simulink model "v2012_DynStab"  (Simulink 7.6)
(part 3 of 4)

      mask prompts: p2_3q "Power and Voltage Ratings [MVA, kV]"; p4_5q "Active and Reactive Powers [p.u.  p.u.]"; p6_7q "Maximum and Minimum Allowable Voltage [p.u.   p.u.]"; p8q "Allow conversion to impendance for min or max voltage"; p9q "Connected"
      mask help:
      | This block defines a constant power load:
      |
      | P = Pcost.
      | Q = Qcost.
      mask CallbackString: |||fm_block|fm_block
      mask Display: plot([1 -0.5 -0.5 1],[0 0.866 -0.866 0])
  PQ23 : PMComponent  Tag=PSATblock  Description=Power Flow  PhysicalDomain=psatdomain  LeftPortType=p1  RightPortType=p1  LConnTagsString=__newl0  mask(PQ){p2_3q=[100 230], p4_5q=[2.2396 1.0847]*1.0722, p6_7q=[1.2  0.8], p8q=off, p9q=on}
      mask prompts: p2_3q "Power and Voltage Ratings [MVA, kV]"; p4_5q "Active and Reactive Powers [p.u.  p.u.]"; p6_7q "Maximum and Minimum Allowable Voltage [p.u.   p.u.]"; p8q "Allow conversion to impendance for min or max voltage"; p9q "Connected"
      mask help:
      | This block defines a constant power load:
      |
      | P = Pcost.
      | Q = Qcost.
      mask CallbackString: |||fm_block|fm_block
      mask Display: plot([1 -0.5 -0.5 1],[0 0.866 -0.866 0])
  PQ24 : PMComponent  Tag=PSATblock  Description=Power Flow  PhysicalDomain=psatdomain  LeftPortType=p1  RightPortType=p1  LConnTagsString=__newl0  mask(PQ){p2_3q=[100  230], p4_5q=[0.3089 0.1697]*1.0722, p6_7q=[1.2  0.8], p8q=off, p9q=on}
      mask prompts: p2_3q "Power and Voltage Ratings [MVA, kV]"; p4_5q "Active and Reactive Powers [p.u.  p.u.]"; p6_7q "Maximum and Minimum Allowable Voltage [p.u.   p.u.]"; p8q "Allow conversion to impendance for min or max voltage"; p9q "Connected"
      mask help:
      | This block defines a constant power load:
      |
      | P = Pcost.
      | Q = Qcost.
      mask CallbackString: |||fm_block|fm_block
      mask Display: plot([1 -0.5 -0.5 1],[0 0.866 -0.866 0])
  PQ25 : PMComponent  Tag=PSATblock  Description=Power Flow  PhysicalDomain=psatdomain  LeftPortType=p1  RightPortType=p1  LConnTagsString=__newl0  mask(PQ){p2_3q=[100  230], p4_5q=[0.1545 0.0848]*1.0722, p6_7q=[1.2  0.8], p8q=off, p9q=on}
      mask prompts: p2_3q "Power and Voltage Ratings [MVA, kV]"; p4_5q "Active and Reactive Powers [p.u.  p.u.]"; p6_7q "Maximum and Minimum Allowable Voltage [p.u.   p.u.]"; p8q "Allow conversion to impendance for min or max voltage"; p9q "Connected"
      mask help:
      | This block defines a constant power load:
      |
      | P = Pcost.
      | Q = Qcost.
      mask CallbackString: |||fm_block|fm_block
      mask Display: plot([1 -0.5 -0.5 1],[0 0.866 -0.866 0])
  PQ26 : PMComponent  Tag=PSATblock  Description=Power Flow  PhysicalDomain=psatdomain  LeftPortType=p1  RightPortType=p1  LConnTagsString=__newl0  mask(PQ){p2_3q=[100  230], p4_5q=[1.0497 0.5401]*1.0722, p6_7q=[1.2  0.8], p8q=off, p9q=on}
      mask prompts: p2_3q "Power and Voltage Ratings [MVA, kV]"; p4_5q "Active and Reactive Powers [p.u.  p.u.]"; p6_7q "Maximum and Minimum Allowable Voltage [p.u.   p.u.]"; p8q "Allow conversion to impendance for min or max voltage"; p9q "Connected"
      mask help:
      | This block defines a constant power load:
      |
      | P = Pcost.
      | Q = Qcost.
      mask CallbackString: |||fm_block|fm_block
      mask Display: plot([1 -0.5 -0.5 1],[0 0.866 -0.866 0])
  PQ27 : PMComponent  Tag=PSATblock  Description=Power Flow  PhysicalDomain=psatdomain  LeftPortType=p1  RightPortType=p1  LConnTagsString=__newl0  mask(PQ){p2_3q=[100 230], p4_5q=[3.7115 1.8795]*1.0722, p6_7q=[1.2  0.8], p8q=off, p9q=on}
      mask prompts: p2_3q "Power and Voltage Ratings [MVA, kV]"; p4_5q "Active and Reactive Powers [p.u.  p.u.]"; p6_7q "Maximum and Minimum Allowable Voltage [p.u.   p.u.]"; p8q "Allow conversion to impendance for min or max voltage"; p9q "Connected"
      mask help:
      | This block defines a constant power load:
      |
      | P = Pcost.
      | Q = Qcost.
      mask CallbackString: |||fm_block|fm_block
      mask Display: plot([1 -0.5 -0.5 1],[0 0.866 -0.866 0])
  PQ28 : PMComponent  Tag=PSATblock  Description=Power Flow  PhysicalDomain=psatdomain  LeftPortType=p1  RightPortType=p1  LConnTagsString=__newl0  mask(PQ){p2_3q=[100 400], p4_5q=[0.5245 0.3107]*1.0722, p6_7q=[1.2  0.8], p8q=off, p9q=on}
      mask prompts: p2_3q "Power and Voltage Ratings [MVA, kV]"; p4_5q "Active and Reactive Powers [p.u.  p.u.]"; p6_7q "Maximum and Minimum Allowable Voltage [p.u.   p.u.]"; p8q "Allow conversion to impendance for min or max voltage"; p9q "Connected"
      mask help:
      | This block defines a constant power load:
      |
      | P = Pcost.
      | Q = Qcost.
      mask CallbackString: |||fm_block|fm_block
      mask Display: plot([1 -0.5 -0.5 1],[0 0.866 -0.866 0])
  PQ29 : PMComponent  Tag=PSATblock  Description=Power Flow  PhysicalDomain=psatdomain  LeftPortType=p1  RightPortType=p1  LConnTagsString=__newl0  mask(PQ){p2_3q=[100 230], p4_5q=[3.0188 1.4621]*1.0722, p6_7q=[1.2  0.8], p8q=off, p9q=on}
      mask prompts: p2_3q "Power and Voltage Ratings [MVA, kV]"; p4_5q "Active and Reactive Powers [p.u.  p.u.]"; p6_7q "Maximum and Minimum Allowable Voltage [p.u.   p.u.]"; p8q "Allow conversion to impendance for min or max voltage"; p9q "Connected"
      mask help:
      | This block defines a constant power load:
      |
      | P = Pcost.
      | Q = Qcost.
      mask CallbackString: |||fm_block|fm_block
      mask Display: plot([1 -0.5 -0.5 1],[0 0.866 -0.866 0])
  PQ3 : PMComponent  Tag=PSATblock  Description=Power Flow  PhysicalDomain=psatdomain  LeftPortType=p1  RightPortType=p1  LConnTagsString=__newl0  mask(PQ){p2_3q=[100 230], p4_5q=[0.3718 0.229]*1.0722, p6_7q=[1.2  0.8], p8q=off, p9q=on}
      mask prompts: p2_3q "Power and Voltage Ratings [MVA, kV]"; p4_5q "Active and Reactive Powers [p.u.  p.u.]"; p6_7q "Maximum and Minimum Allowable Voltage [p.u.   p.u.]"; p8q "Allow conversion to impendance for min or max voltage"; p9q "Connected"
      mask help:
      | This block defines a constant power load:
      |
      | P = Pcost.
      | Q = Qcost.
      mask CallbackString: |||fm_block|fm_block
      mask Display: plot([1 -0.5 -0.5 1],[0 0.866 -0.866 0])
  PQ30 : PMComponent  Tag=PSATblock  Description=Power Flow  PhysicalDomain=psatdomain  LeftPortType=p1  RightPortType=p1  LConnTagsString=__newl0  mask(PQ){p2_3q=[100 400], p4_5q=[0.9057 0.4386]*1.0722, p6_7q=[1.2  0.8], p8q=off, p9q=on}
      mask prompts: p2_3q "Power and Voltage Ratings [MVA, kV]"; p4_5q "Active and Reactive Powers [p.u.  p.u.]"; p6_7q "Maximum and Minimum Allowable Voltage [p.u.   p.u.]"; p8q "Allow conversion to impendance for min or max voltage"; p9q "Connected"
      mask help:
      | This block defines a constant power load:
      |
      | P = Pcost.
      | Q = Qcost.
      mask CallbackString: |||fm_block|fm_block
      mask Display: plot([1 -0.5 -0.5 1],[0 0.866 -0.866 0])
  PQ31 : PMComponent  Tag=PSATblock  Description=Power Flow  PhysicalDomain=psatdomain  LeftPortType=p1  RightPortType=p1  LConnTagsString=__newl0  mask(PQ){p2_3q=[100 400], p4_5q=[3.0188 1.4621]*1.0722, p6_7q=[1.2  0.8], p8q=off, p9q=on}
      mask prompts: p2_3q "Power and Voltage Ratings [MVA, kV]"; p4_5q "Active and Reactive Powers [p.u.  p.u.]"; p6_7q "Maximum and Minimum Allowable Voltage [p.u.   p.u.]"; p8q "Allow conversion to impendance for min or max voltage"; p9q "Connected"
      mask help:
      | This block defines a constant power load:
      |
      | P = Pcost.
      | Q = Qcost.
      mask CallbackString: |||fm_block|fm_block
      mask Display: plot([1 -0.5 -0.5 1],[0 0.866 -0.866 0])
  PQ32 : PMComponent  Tag=PSATblock  Description=Power Flow  PhysicalDomain=psatdomain  LeftPortType=p1  RightPortType=p1  LConnTagsString=__newl0  mask(PQ){p2_3q=[100 230], p4_5q=[2.2641 1.0966]*1.0722, p6_7q=[1.2  0.8], p8q=off, p9q=on}
      mask prompts: p2_3q "Power and Voltage Ratings [MVA, kV]"; p4_5q "Active and Reactive Powers [p.u.  p.u.]"; p6_7q "Maximum and Minimum Allowable Voltage [p.u.   p.u.]"; p8q "Allow conversion to impendance for min or max voltage"; p9q "Connected"
      mask help:
      | This block defines a constant power load:
      |
      | P = Pcost.
      | Q = Qcost.
      mask CallbackString: |||fm_block|fm_block
      mask Display: plot([1 -0.5 -0.5 1],[0 0.866 -0.866 0])
  PQ33 : PMComponent  Tag=PSATblock  Description=Power Flow  PhysicalDomain=psatdomain  LeftPortType=p1  RightPortType=p1  LConnTagsString=__newl0  mask(PQ){p2_3q=[100 400], p4_5q=[1.8752 1.3089]*1.0722, p6_7q=[1.2  0.8], p8q=off, p9q=on}
      mask prompts: p2_3q "Power and Voltage Ratings [MVA, kV]"; p4_5q "Active and Reactive Powers [p.u.  p.u.]"; p6_7q "Maximum and Minimum Allowable Voltage [p.u.   p.u.]"; p8q "Allow conversion to impendance for min or max voltage"; p9q "Connected"
      mask help:
      | This block defines a constant power load:
      |
      | P = Pcost.
      | Q = Qcost.
      mask CallbackString: |||fm_block|fm_block
      mask Display: plot([1 -0.5 -0.5 1],[0 0.866 -0.866 0])
  PQ34 : PMComponent  Tag=PSATblock  Description=Power Flow  PhysicalDomain=psatdomain  LeftPortType=p1  RightPortType=p1  LConnTagsString=__newl0  mask(PQ){p2_3q=[100 230], p4_5q=[0.2843 0.2054]*1.0722, p6_7q=[1.2  0.8], p8q=off, p9q=on}
      mask prompts: p2_3q "Power and Voltage Ratings [MVA, kV]"; p4_5q "Active and Reactive Powers [p.u.  p.u.]"; p6_7q "Maximum and Minimum Allowable Voltage [p.u.   p.u.]"; p8q "Allow conversion to impendance for min or max voltage"; p9q "Connected"
      mask help:
      | This block defines a constant power load:
      |
      | P = Pcost.
      | Q = Qcost.
      mask CallbackString: |||fm_block|fm_block
      mask Display: plot([1 -0.5 -0.5 1],[0 0.866 -0.866 0])
  PQ35 : PMComponent  Tag=PSATblock  Description=Power Flow  PhysicalDomain=psatdomain  LeftPortType=p1  RightPortType=p1  LConnTagsString=__newl0  mask(PQ){p2_3q=[100 230], p4_5q=[0.2843 0.2054]*1.0722, p6_7q=[1.2  0.8], p8q=off, p9q=on}
      mask prompts: p2_3q "Power and Voltage Ratings [MVA, kV]"; p4_5q "Active and Reactive Powers [p.u.  p.u.]"; p6_7q "Maximum and Minimum Allowable Voltage [p.u.   p.u.]"; p8q "Allow conversion to impendance for min or max voltage"; p9q "Connected"
      mask help:
      | This block defines a constant power load:
      |
      | P = Pcost.
      | Q = Qcost.
      mask CallbackString: |||fm_block|fm_block
      mask Display: plot([1 -0.5 -0.5 1],[0 0.866 -0.866 0])
  PQ36 : PMComponent  Tag=PSATblock  Description=Power Flow  PhysicalDomain=psatdomain  LeftPortType=p1  RightPortType=p1  LConnTagsString=__newl0  mask(PQ){p2_3q=[100 400], p4_5q=[36.6028 17.7846]*1.0722, p6_7q=[1.2  0.8], p8q=off, p9q=on}
      mask prompts: p2_3q "Power and Voltage Ratings [MVA, kV]"; p4_5q "Active and Reactive Powers [p.u.  p.u.]"; p6_7q "Maximum and Minimum Allowable Voltage [p.u.   p.u.]"; p8q "Allow conversion to impendance for min or max voltage"; p9q "Connected"
      mask help:
      | This block defines a constant power load:
      |
      | P = Pcost.
      | Q = Qcost.
      mask CallbackString: |||fm_block|fm_block
      mask Display: plot([1 -0.5 -0.5 1],[0 0.866 -0.866 0])
  PQ37 : PMComponent  Tag=PSATblock  Description=Power Flow  PhysicalDomain=psatdomain  LeftPortType=p1  RightPortType=p1  LConnTagsString=__newl0  mask(PQ){p2_3q=[100  138], p4_5q=[1.6201 0.7847]*1.0722, p6_7q=[1.2  0.8], p8q=off, p9q=on}
      mask prompts: p2_3q "Power and Voltage Ratings [MVA, kV]"; p4_5q "Active and Reactive Powers [p.u.  p.u.]"; p6_7q "Maximum and Minimum Allowable Voltage [p.u.   p.u.]"; p8q "Allow conversion to impendance for min or max voltage"; p9q "Connected"
      mask help:
      | This block defines a constant power load:
      |
      | P = Pcost.
      | Q = Qcost.
      mask CallbackString: |||fm_block|fm_block
      mask Display: plot([1 -0.5 -0.5 1],[0 0.866 -0.866 0])
  PQ38 : PMComponent  Tag=PSATblock  Description=Power Flow  PhysicalDomain=psatdomain  LeftPortType=p1  RightPortType=p1  LConnTagsString=__newl0  mask(PQ){p2_3q=[100  230], p4_5q=[0.5061 0.2587]*1.0722, p6_7q=[1.2  0.8], p8q=off, p9q=on}
      mask prompts: p2_3q "Power and Voltage Ratings [MVA, kV]"; p4_5q "Active and Reactive Powers [p.u.  p.u.]"; p6_7q "Maximum and Minimum Allowable Voltage [p.u.   p.u.]"; p8q "Allow conversion to impendance for min or max voltage"; p9q "Connected"
      mask help:
      | This block defines a constant power load:
      |
      | P = Pcost.
      | Q = Qcost.
      mask CallbackString: |||fm_block|fm_block
      mask Display: plot([1 -0.5 -0.5 1],[0 0.866 -0.866 0])
  PQ39 : PMComponent  Tag=PSATblock  Description=Power Flow  PhysicalDomain=psatdomain  LeftPortType=p1  RightPortType=p1  LConnTagsString=__newl0  mask(PQ){p2_3q=[100 230], p4_5q=[3.5335 1.7114]*1.0722, p6_7q=[1.2  0.8], p8q=off, p9q=on}
      mask prompts: p2_3q "Power and Voltage Ratings [MVA, kV]"; p4_5q "Active and Reactive Powers [p.u.  p.u.]"; p6_7q "Maximum and Minimum Allowable Voltage [p.u.   p.u.]"; p8q "Allow conversion to impendance for min or max voltage"; p9q "Connected"
      mask help:
      | This block defines a constant power load:
      |
      | P = Pcost.
      | Q = Qcost.
      mask CallbackString: |||fm_block|fm_block
      mask Display: plot([1 -0.5 -0.5 1],[0 0.866 -0.866 0])
  PQ4 : PMComponent  Tag=PSATblock  Description=Power Flow  PhysicalDomain=psatdomain  LeftPortType=p1  RightPortType=p1  LConnTagsString=__newl0  mask(PQ){p2_3q=[100 765], p4_5q=[0.0488 19.5074], p6_7q=[1.2  0.8], p8q=off, p9q=on}
      mask prompts: p2_3q "Power and Voltage Ratings [MVA, kV]"; p4_5q "Active and Reactive Powers [p.u.  p.u.]"; p6_7q "Maximum and Minimum Allowable Voltage [p.u.   p.u.]"; p8q "Allow conversion to impendance for min or max voltage"; p9q "Connected"
      mask help:
      | This block defines a constant power load:
      |
      | P = Pcost.
      | Q = Qcost.
      mask CallbackString: |||fm_block|fm_block
      mask Display: plot([1 -0.5 -0.5 1],[0 0.866 -0.866 0])
  PQ40 : PMComponent  Tag=PSATblock  Description=Power Flow  PhysicalDomain=psatdomain  LeftPortType=p1  RightPortType=p1  LConnTagsString=__newl0  mask(PQ){p2_3q=[100 230], p4_5q=[2.3557 1.1409]*1.0722, p6_7q=[1.2  0.8], p8q=off, p9q=on}
      mask prompts: p2_3q "Power and Voltage Ratings [MVA, kV]"; p4_5q "Active and Reactive Powers [p.u.  p.u.]"; p6_7q "Maximum and Minimum Allowable Voltage [p.u.   p.u.]"; p8q "Allow conversion to impendance for min or max voltage"; p9q "Connected"
      mask help:
      | This block defines a constant power load:
      |
      | P = Pcost.
      | Q = Qcost.
      mask CallbackString: |||fm_block|fm_block
      mask Display: plot([1 -0.5 -0.5 1],[0 0.866 -0.866 0])
  PQ41 : PMComponent  Tag=PSATblock  Description=Power Flow  PhysicalDomain=psatdomain  LeftPortType=p1  RightPortType=p1  LConnTagsString=__newl0  mask(PQ){p2_3q=[100 230], p4_5q=[3.5335 1.7114]*1.0722, p6_7q=[1.2  0.8], p8q=off, p9q=on}
      mask prompts: p2_3q "Power and Voltage Ratings [MVA, kV]"; p4_5q "Active and Reactive Powers [p.u.  p.u.]"; p6_7q "Maximum and Minimum Allowable Voltage [p.u.   p.u.]"; p8q "Allow conversion to impendance for min or max voltage"; p9q "Connected"
      mask help:
      | This block defines a constant power load:
      |
      | P = Pcost.
      | Q = Qcost.
      mask CallbackString: |||fm_block|fm_block
      mask Display: plot([1 -0.5 -0.5 1],[0 0.866 -0.866 0])
  PQ42 : PMComponent  Tag=PSATblock  Description=Power Flow  PhysicalDomain=psatdomain  LeftPortType=p1  RightPortType=p1  LConnTagsString=__newl0  mask(PQ){p2_3q=[100 230], p4_5q=[2.3557 1.1409]*1.0722, p6_7q=[1.2  0.8], p8q=off, p9q=on}
      mask prompts: p2_3q "Power and Voltage Ratings [MVA, kV]"; p4_5q "Active and Reactive Powers [p.u.  p.u.]"; p6_7q "Maximum and Minimum Allowable Voltage [p.u.   p.u.]"; p8q "Allow conversion to impendance for min or max voltage"; p9q "Connected"
      mask help:
      | This block defines a constant power load:
      |
      | P = Pcost.
      | Q = Qcost.
      mask CallbackString: |||fm_block|fm_block
      mask Display: plot([1 -0.5 -0.5 1],[0 0.866 -0.866 0])
  PQ43 : PMComponent  Tag=PSATblock  Description=Power Flow  PhysicalDomain=psatdomain  LeftPortType=p1  RightPortType=p1  LConnTagsString=__newl0  mask(PQ){p2_3q=[100 765], p4_5q=[0.0122 4.8769]*1.0722, p6_7q=[1.2  0.8], p8q=off, p9q=on}
      mask prompts: p2_3q "Power and Voltage Ratings [MVA, kV]"; p4_5q "Active and Reactive Powers [p.u.  p.u.]"; p6_7q "Maximum and Minimum Allowable Voltage [p.u.   p.u.]"; p8q "Allow conversion to impendance for min or max voltage"; p9q "Connected"
      mask help:
      | This block defines a constant power load:
      |
      | P = Pcost.
      | Q = Qcost.
      mask CallbackString: |||fm_block|fm_block
      mask Display: plot([1 -0.5 -0.5 1],[0 0.866 -0.866 0])
  PQ44 : PMComponent  Tag=PSATblock  Description=Power Flow  PhysicalDomain=psatdomain  LeftPortType=p1  RightPortType=p1  LConnTagsString=__newl0  mask(PQ){p2_3q=[100 230], p4_5q=[5.8892 2.8523]*1.0722, p6_7q=[1.2  0.8], p8q=off, p9q=on}
      mask prompts: p2_3q "Power and Voltage Ratings [MVA, kV]"; p4_5q "Active and Reactive Powers [p.u.  p.u.]"; p6_7q "Maximum and Minimum Allowable Voltage [p.u.   p.u.]"; p8q "Allow conversion to impendance for min or max voltage"; p9q "Connected"
      mask help:
      | This block defines a constant power load:
      |
      | P = Pcost.
      | Q = Qcost.
      mask CallbackString: |||fm_block|fm_block
      mask Display: plot([1 -0.5 -0.5 1],[0 0.866 -0.866 0])
  PQ45 : PMComponent  Tag=PSATblock  Description=Power Flow  PhysicalDomain=psatdomain  LeftPortType=p1  RightPortType=p1  LConnTagsString=__newl0  mask(PQ){p2_3q=[100  230], p4_5q=[0.6*3.7739 0.6*1.8278]*1.0722, p6_7q=[1.2  0.8], p8q=off, p9q=on}
      mask prompts: p2_3q "Power and Voltage Ratings [MVA, kV]"; p4_5q "Active and Reactive Powers [p.u.  p.u.]"; p6_7q "Maximum and Minimum Allowable Voltage [p.u.   p.u.]"; p8q "Allow conversion to impendance for min or max voltage"; p9q "Connected"
      mask help:
      | This block defines a constant power load:
      |
      | P = Pcost.
      | Q = Qcost.
      mask CallbackString: |||fm_block|fm_block
      mask Display: plot([1 -0.5 -0.5 1],[0 0.866 -0.866 0])
  PQ46 : PMComponent  Tag=PSATblock  Description=Power Flow  PhysicalDomain=psatdomain  LeftPortType=p1  RightPortType=p1  LConnTagsString=__newl0  mask(PQ){p2_3q=[100 765], p4_5q=[0.0163 6.5025], p6_7q=[1.2  0.8], p8q=off, p9q=on}
      mask prompts: p2_3q "Power and Voltage Ratings [MVA, kV]"; p4_5q "Active and Reactive Powers [p.u.  p.u.]"; p6_7q "Maximum and Minimum Allowable Voltage [p.u.   p.u.]"; p8q "Allow conversion to impendance for min or max voltage"; p9q "Connected"
      mask help:
      | This block defines a constant power load:
      |
      | P = Pcost.
      | Q = Qcost.
      mask CallbackString: |||fm_block|fm_block
      mask Display: plot([1 -0.5 -0.5 1],[0 0.866 -0.866 0])
  PQ47 : PMComponent  Tag=PSATblock  Description=Power Flow  PhysicalDomain=psatdomain  LeftPortType=p1  RightPortType=p1  LConnTagsString=__newl0  mask(PQ){p2_3q=[100 115], p4_5q=[1.5322*0.3 0.7421*0.3]*1.0722, p6_7q=[1.2  0.8], p8q=off, p9q=on}
      mask prompts: p2_3q "Power and Voltage Ratings [MVA, kV]"; p4_5q "Active and Reactive Powers [p.u.  p.u.]"; p6_7q "Maximum and Minimum Allowable Voltage [p.u.   p.u.]"; p8q "Allow conversion to impendance for min or max voltage"; p9q "Connected"
      mask help:
      | This block defines a constant power load:
      |
      | P = Pcost.
      | Q = Qcost.
      mask CallbackString: |||fm_block|fm_block
      mask Display: plot([1 -0.5 -0.5 1],[0 0.866 -0.866 0])
  PQ48 : PMComponent  Tag=PSATblock  Description=Power Flow  PhysicalDomain=psatdomain  LeftPortType=p1  RightPortType=p1  LConnTagsString=__newl0  mask(PQ){p2_3q=[100 230], p4_5q=[0.1160 0.0562]*1.0722, p6_7q=[1.2  0.8], p8q=off, p9q=on}
      mask prompts: p2_3q "Power and Voltage Ratings [MVA, kV]"; p4_5q "Active and Reactive Powers [p.u.  p.u.]"; p6_7q "Maximum and Minimum Allowable Voltage [p.u.   p.u.]"; p8q "Allow conversion to impendance for min or max voltage"; p9q "Connected"
      mask help:
      | This block defines a constant power load:
      |
      | P = Pcost.
      | Q = Qcost.
      mask CallbackString: |||fm_block|fm_block
      mask Display: plot([1 -0.5 -0.5 1],[0 0.866 -0.866 0])
  PQ49 : PMComponent  Tag=PSATblock  Description=Power Flow  PhysicalDomain=psatdomain  LeftPortType=p1  RightPortType=p1  LConnTagsString=__newl0  mask(PQ){p2_3q=[100 230], p4_5q=[0.9861 0.4776]*1.0722, p6_7q=[1.2  0.8], p8q=off, p9q=on}
      mask prompts: p2_3q "Power and Voltage Ratings [MVA, kV]"; p4_5q "Active and Reactive Powers [p.u.  p.u.]"; p6_7q "Maximum and Minimum Allowable Voltage [p.u.   p.u.]"; p8q "Allow conversion to impendance for min or max voltage"; p9q "Connected"
      mask help:
      | This block defines a constant power load:
      |
      | P = Pcost.
      | Q = Qcost.
      mask CallbackString: |||fm_block|fm_block
      mask Display: plot([1 -0.5 -0.5 1],[0 0.866 -0.866 0])
  PQ5 : PMComponent  Tag=PSATblock  Description=Power Flow  PhysicalDomain=psatdomain  LeftPortType=p1  RightPortType=p1  LConnTagsString=__newl0  mask(PQ){p2_3q=[100  230], p4_5q=[2.9191 1.4138]*1.0722, p6_7q=[1.2  0.8], p8q=off, p9q=on}
      mask prompts: p2_3q "Power and Voltage Ratings [MVA, kV]"; p4_5q "Active and Reactive Powers [p.u.  p.u.]"; p6_7q "Maximum and Minimum Allowable Voltage [p.u.   p.u.]"; p8q "Allow conversion to impendance for min or max voltage"; p9q "Connected"
      mask help:
      | This block defines a constant power load:
      |
      | P = Pcost.
      | Q = Qcost.
      mask CallbackString: |||fm_block|fm_block
      mask Display: plot([1 -0.5 -0.5 1],[0 0.866 -0.866 0])
  PQ50 : PMComponent  Tag=PSATblock  Description=Power Flow  PhysicalDomain=psatdomain  LeftPortType=p1  RightPortType=p1  LConnTagsString=__newl0  mask(PQ){p2_3q=[100  115], p4_5q=[3.7739*0.2 1.8278*0.2]*1.0722, p6_7q=[1.2  0.8], p8q=off, p9q=on}
      mask prompts: p2_3q "Power and Voltage Ratings [MVA, kV]"; p4_5q "Active and Reactive Powers [p.u.  p.u.]"; p6_7q "Maximum and Minimum Allowable Voltage [p.u.   p.u.]"; p8q "Allow conversion to impendance for min or max voltage"; p9q "Connected"
      mask help:
      | This block defines a constant power load:
      |
      | P = Pcost.
      | Q = Qcost.
      mask CallbackString: |||fm_block|fm_block
      mask Display: plot([1 -0.5 -0.5 1],[0 0.866 -0.866 0])
  PQ51 : PMComponent  Tag=PSATblock  Description=Power Flow  PhysicalDomain=psatdomain  LeftPortType=p1  RightPortType=p1  LConnTagsString=__newl0  mask(PQ){p2_3q=[100  138], p4_5q=[4.6365 2.2456]*1.0722, p6_7q=[1.2  0.8], p8q=off, p9q=on}
      mask prompts: p2_3q "Power and Voltage Ratings [MVA, kV]"; p4_5q "Active and Reactive Powers [p.u.  p.u.]"; p6_7q "Maximum and Minimum Allowable Voltage [p.u.   p.u.]"; p8q "Allow conversion to impendance for min or max voltage"; p9q "Connected"
      mask help:
      | This block defines a constant power load:
      |
      | P = Pcost.
      | Q = Qcost.
      mask CallbackString: |||fm_block|fm_block
      mask Display: plot([1 -0.5 -0.5 1],[0 0.866 -0.866 0])
  PQ52 : PMComponent  Tag=PSATblock  Description=Power Flow  PhysicalDomain=psatdomain  LeftPortType=p1  RightPortType=p1  LConnTagsString=__newl0  mask(PQ){p2_3q=[100  138], p4_5q=[1.6201 0.7847]*1.0722, p6_7q=[1.2  0.8], p8q=off, p9q=on}
      mask prompts: p2_3q "Power and Voltage Ratings [MVA, kV]"; p4_5q "Active and Reactive Powers [p.u.  p.u.]"; p6_7q "Maximum and Minimum Allowable Voltage [p.u.   p.u.]"; p8q "Allow conversion to impendance for min or max voltage"; p9q "Connected"
      mask help:
      | This block defines a constant power load:
      |
      | P = Pcost.
      | Q = Qcost.
      mask CallbackString: |||fm_block|fm_block
      mask Display: plot([1 -0.5 -0.5 1],[0 0.866 -0.866 0])
  PQ53 : PMComponent  Tag=PSATblock  Description=Power Flow  PhysicalDomain=psatdomain  LeftPortType=p1  RightPortType=p1  LConnTagsString=__newl0  mask(PQ){p2_3q=[100  138], p4_5q=[1.6201 0.7847]*1.0722, p6_7q=[1.2  0.8], p8q=off, p9q=on}
      mask prompts: p2_3q "Power and Voltage Ratings [MVA, kV]"; p4_5q "Active and Reactive Powers [p.u.  p.u.]"; p6_7q "Maximum and Minimum Allowable Voltage [p.u.   p.u.]"; p8q "Allow conversion to impendance for min or max voltage"; p9q "Connected"
      mask help:
      | This block defines a constant power load:
      |
      | P = Pcost.
      | Q = Qcost.
      mask CallbackString: |||fm_block|fm_block
      mask Display: plot([1 -0.5 -0.5 1],[0 0.866 -0.866 0])
  PQ54 : PMComponent  Tag=PSATblock  Description=Power Flow  PhysicalDomain=psatdomain  LeftPortType=p1  RightPortType=p1  LConnTagsString=__newl0  mask(PQ){p2_3q=[100  138], p4_5q=[1.6201 0.7847]*1.0722, p6_7q=[1.2  0.8], p8q=off, p9q=on}
      mask prompts: p2_3q "Power and Voltage Ratings [MVA, kV]"; p4_5q "Active and Reactive Powers [p.u.  p.u.]"; p6_7q "Maximum and Minimum Allowable Voltage [p.u.   p.u.]"; p8q "Allow conversion to impendance for min or max voltage"; p9q "Connected"
      mask help:
      | This block defines a constant power load:
      |
      | P = Pcost.
      | Q = Qcost.
      mask CallbackString: |||fm_block|fm_block
      mask Display: plot([1 -0.5 -0.5 1],[0 0.866 -0.866 0])
  PQ55 : PMComponent  Tag=PSATblock  Description=Power Flow  PhysicalDomain=psatdomain  LeftPortType=p1  RightPortType=p1  LConnTagsString=__newl0  mask(PQ){p2_3q=[100  138], p4_5q=[8.3216 4.0303]*1.0722, p6_7q=[1.2  0.8], p8q=off, p9q=on}
      mask prompts: p2_3q "Power and Voltage Ratings [MVA, kV]"; p4_5q "Active and Reactive Powers [p.u.  p.u.]"; p6_7q "Maximum and Minimum Allowable Voltage [p.u.   p.u.]"; p8q "Allow conversion to impendance for min or max voltage"; p9q "Connected"
      mask help:
      | This block defines a constant power load:
      |
      | P = Pcost.
      | Q = Qcost.
      mask CallbackString: |||fm_block|fm_block
      mask Display: plot([1 -0.5 -0.5 1],[0 0.866 -0.866 0])
  PQ56 : PMComponent  Tag=PSATblock  Description=Power Flow  PhysicalDomain=psatdomain  LeftPortType=p1  RightPortType=p1  LConnTagsString=__newl0  mask(PQ){p2_3q=[100  115], p4_5q=[3.7739*0.2 1.8278*0.2]*1.0722, p6_7q=[1.2  0.8], p8q=off, p9q=on}
      mask prompts: p2_3q "Power and Voltage Ratings [MVA, kV]"; p4_5q "Active and Reactive Powers [p.u.  p.u.]"; p6_7q "Maximum and Minimum Allowable Voltage [p.u.   p.u.]"; p8q "Allow conversion to impendance for min or max voltage"; p9q "Connected"
      mask help:
      | This block defines a constant power load:
      |
      | P = Pcost.
      | Q = Qcost.
      mask CallbackString: |||fm_block|fm_block
      mask Display: plot([1 -0.5 -0.5 1],[0 0.866 -0.866 0])
  PQ57 : PMComponent  Tag=PSATblock  Description=Power Flow  PhysicalDomain=psatdomain  LeftPortType=p1  RightPortType=p1  LConnTagsString=__newl0  mask(PQ){p2_3q=[100 115], p4_5q=[1.0215*0.25 0.4947*0.25]*1.0722, p6_7q=[1.2  0.8], p8q=off, p9q=on}
      mask prompts: p2_3q "Power and Voltage Ratings [MVA, kV]"; p4_5q "Active and Reactive Powers [p.u.  p.u.]"; p6_7q "Maximum and Minimum Allowable Voltage [p.u.   p.u.]"; p8q "Allow conversion to impendance for min or max voltage"; p9q "Connected"
      mask help:
      | This block defines a constant power load:
      |
      | P = Pcost.
      | Q = Qcost.
      mask CallbackString: |||fm_block|fm_block
      mask Display: plot([1 -0.5 -0.5 1],[0 0.866 -0.866 0])
  PQ58 : PMComponent  Tag=PSATblock  Description=Power Flow  PhysicalDomain=psatdomain  LeftPortType=p1  RightPortType=p1  LConnTagsString=__newl0  mask(PQ){p2_3q=[100  230], p4_5q=[0.0264 10.58], p6_7q=[1.2  0.8], p8q=off, p9q=off}
      mask prompts: p2_3q "Power and Voltage Ratings [MVA, kV]"; p4_5q "Active and Reactive Powers [p.u.  p.u.]"; p6_7q "Maximum and Minimum Allowable Voltage [p.u.   p.u.]"; p8q "Allow conversion to impendance for min or max voltage"; p9q "Connected"
      mask help:
      | This block defines a constant power load:
      |
      | P = Pcost.
      | Q = Qcost.
      mask CallbackString: |||fm_block|fm_block
      mask Display: plot([1 -0.5 -0.5 1],[0 0.866 -0.866 0])
  PQ59 : PMComponent  Tag=PSATblock  Description=Power Flow  PhysicalDomain=psatdomain  LeftPortType=p1  RightPortType=p1  LConnTagsString=__newl0  mask(PQ){p2_3q=[100  230], p4_5q=[0.0264 10.58], p6_7q=[1.2  0.8], p8q=off, p9q=off}
      mask prompts: p2_3q "Power and Voltage Ratings [MVA, kV]"; p4_5q "Active and Reactive Powers [p.u.  p.u.]"; p6_7q "Maximum and Minimum Allowable Voltage [p.u.   p.u.]"; p8q "Allow conversion to impendance for min or max voltage"; p9q "Connected"
      mask help:
      | This block defines a constant power load:
      |
      | P = Pcost.
      | Q = Qcost.
      mask CallbackString: |||fm_block|fm_block
      mask Display: plot([1 -0.5 -0.5 1],[0 0.866 -0.866 0])
  PQ6 : PMComponent  Tag=PSATblock  Description=Power Flow  PhysicalDomain=psatdomain  LeftPortType=p1  RightPortType=p1  LConnTagsString=__newl0  mask(PQ){p2_3q=[100 230], p4_5q=[0.2898 0.2057]*1.0722, p6_7q=[1.2  0.8], p8q=off, p9q=on}
      mask prompts: p2_3q "Power and Voltage Ratings [MVA, kV]"; p4_5q "Active and Reactive Powers [p.u.  p.u.]"; p6_7q "Maximum and Minimum Allowable Voltage [p.u.   p.u.]"; p8q "Allow conversion to impendance for min or max voltage"; p9q "Connected"
      mask help:
      | This block defines a constant power load:
      |
      | P = Pcost.
      | Q = Qcost.
      mask CallbackString: |||fm_block|fm_block
      mask Display: plot([1 -0.5 -0.5 1],[0 0.866 -0.866 0])
  PQ60 : PMComponent  Tag=PSATblock  Description=Power Flow  PhysicalDomain=psatdomain  LeftPortType=p1  RightPortType=p1  LConnTagsString=__newl0  mask(PQ){p2_3q=[100  230], p4_5q=[0.0264 10.58], p6_7q=[1.2  0.8], p8q=off, p9q=off}
      mask prompts: p2_3q "Power and Voltage Ratings [MVA, kV]"; p4_5q "Active and Reactive Powers [p.u.  p.u.]"; p6_7q "Maximum and Minimum Allowable Voltage [p.u.   p.u.]"; p8q "Allow conversion to impendance for min or max voltage"; p9q "Connected"
      mask help:
      | This block defines a constant power load:
      |
      | P = Pcost.
      | Q = Qcost.
      mask CallbackString: |||fm_block|fm_block
      mask Display: plot([1 -0.5 -0.5 1],[0 0.866 -0.866 0])
  PQ61 : PMComponent  Tag=PSATblock  Description=Power Flow  PhysicalDomain=psatdomain  LeftPortType=p1  RightPortType=p1  LConnTagsString=__newl0  mask(PQ){p2_3q=[100 400], p4_5q=[0.02 8], p6_7q=[1.2  0.8], p8q=off, p9q=off}
      mask prompts: p2_3q "Power and Voltage Ratings [MVA, kV]"; p4_5q "Active and Reactive Powers [p.u.  p.u.]"; p6_7q "Maximum and Minimum Allowable Voltage [p.u.   p.u.]"; p8q "Allow conversion to impendance for min or max voltage"; p9q "Connected"
      mask help:
      | This block defines a constant power load:
      |
      | P = Pcost.
      | Q = Qcost.
      mask CallbackString: |||fm_block|fm_block
      mask Display: plot([1 -0.5 -0.5 1],[0 0.866 -0.866 0])
  PQ62 : PMComponent  Tag=PSATblock  Description=Power Flow  PhysicalDomain=psatdomain  LeftPortType=p1  RightPortType=p1  LConnTagsString=__newl0  mask(PQ){p2_3q=[100 400], p4_5q=[0.02 8], p6_7q=[1.2  0.8], p8q=off, p9q=on}
      mask prompts: p2_3q "Power and Voltage Ratings [MVA, kV]"; p4_5q "Active and Reactive Powers [p.u.  p.u.]"; p6_7q "Maximum and Minimum Allowable Voltage [p.u.   p.u.]"; p8q "Allow conversion to impendance for min or max voltage"; p9q "Connected"
      mask help:
      | This block defines a constant power load:
      |
      | P = Pcost.
      | Q = Qcost.
      mask CallbackString: |||fm_block|fm_block
      mask Display: plot([1 -0.5 -0.5 1],[0 0.866 -0.866 0])
  PQ63 : PMComponent  Tag=PSATblock  Description=Power Flow  PhysicalDomain=psatdomain  LeftPortType=p1  RightPortType=p1  LConnTagsString=__newl0  mask(PQ){p2_3q=[100 400], p4_5q=[0.02 8], p6_7q=[1.2  0.8], p8q=off, p9q=off}
      mask prompts: p2_3q "Power and Voltage Ratings [MVA, kV]"; p4_5q "Active and Reactive Powers [p.u.  p.u.]"; p6_7q "Maximum and Minimum Allowable Voltage [p.u.   p.u.]"; p8q "Allow conversion to impendance for min or max voltage"; p9q "Connected"
      mask help:
      | This block defines a constant power load:
      |
      | P = Pcost.
      | Q = Qcost.
      mask CallbackString: |||fm_block|fm_block
      mask Display: plot([1 -0.5 -0.5 1],[0 0.866 -0.866 0])
  PQ64 : PMComponent  Tag=PSATblock  Description=Power Flow  PhysicalDomain=psatdomain  LeftPortType=p1  RightPortType=p1  LConnTagsString=__newl0  mask(PQ){p2_3q=[1322.5  230], p4_5q=[0.0331 13.2250], p6_7q=[1.2  0.8], p8q=off, p9q=off}
      mask prompts: p2_3q "Power and Voltage Ratings [MVA, kV]"; p4_5q "Active and Reactive Powers [p.u.  p.u.]"; p6_7q "Maximum and Minimum Allowable Voltage [p.u.   p.u.]"; p8q "Allow conversion to impendance for min or max voltage"; p9q "Connected"
      mask help:
      | This block defines a constant power load:
      |
      | P = Pcost.
      | Q = Qcost.
      mask CallbackString: |||fm_block|fm_block
      mask Display: plot([1 -0.5 -0.5 1],[0 0.866 -0.866 0])
  PQ65 : PMComponent  Tag=PSATblock  Description=Power Flow  PhysicalDomain=psatdomain  LeftPortType=p1  RightPortType=p1  LConnTagsString=__newl0  mask(PQ){p2_3q=[100  400], p4_5q=[0.08 31.9999], p6_7q=[1.2  0.8], p8q=off, p9q=off}
      mask prompts: p2_3q "Power and Voltage Ratings [MVA, kV]"; p4_5q "Active and Reactive Powers [p.u.  p.u.]"; p6_7q "Maximum and Minimum Allowable Voltage [p.u.   p.u.]"; p8q "Allow conversion to impendance for min or max voltage"; p9q "Connected"
      mask help:
      | This block defines a constant power load:
      |
      | P = Pcost.
      | Q = Qcost.
      mask CallbackString: |||fm_block|fm_block
      mask Display: plot([1 -0.5 -0.5 1],[0 0.866 -0.866 0])
  PQ66 : PMComponent  Tag=PSATblock  Description=Power Flow  PhysicalDomain=psatdomain  LeftPortType=p1  RightPortType=p1  LConnTagsString=__newl0  mask(PQ){p2_3q=[100  400], p4_5q=[0.04 16], p6_7q=[1.2  0.8], p8q=off, p9q=on}
      mask prompts: p2_3q "Power and Voltage Ratings [MVA, kV]"; p4_5q "Active and Reactive Powers [p.u.  p.u.]"; p6_7q "Maximum and Minimum Allowable Voltage [p.u.   p.u.]"; p8q "Allow conversion to impendance for min or max voltage"; p9q "Connected"
      mask help:
      | This block defines a constant power load:
      |
      | P = Pcost.
      | Q = Qcost.
      mask CallbackString: |||fm_block|fm_block
      mask Display: plot([1 -0.5 -0.5 1],[0 0.866 -0.866 0])
  PQ67 : PMComponent  Tag=PSATblock  Description=Power Flow  PhysicalDomain=psatdomain  LeftPortType=p1  RightPortType=p1  LConnTagsString=__newl0  mask(PQ){p2_3q=[100  400], p4_5q=[0.04 16], p6_7q=[1.2  0.8], p8q=on, p9q=off}
      mask prompts: p2_3q "Power and Voltage Ratings [MVA, kV]"; p4_5q "Active and Reactive Powers [p.u.  p.u.]"; p6_7q "Maximum and Minimum Allowable Voltage [p.u.   p.u.]"; p8q "Allow conversion to impendance for min or max voltage"; p9q "Connected"
      mask help:
      | This block defines a constant power load:
      |
      | P = Pcost.
      | Q = Qcost.
      mask CallbackString: |||fm_block|fm_block
      mask Display: plot([1 -0.5 -0.5 1],[0 0.866 -0.866 0])
  PQ68 : PMComponent  Tag=PSATblock  Description=Power Flow  PhysicalDomain=psatdomain  LeftPortType=p1  RightPortType=p1  LConnTagsString=__newl0  mask(PQ){p2_3q=[100 230], p4_5q=[0.0132 5.29], p6_7q=[1.2  0.8], p8q=off, p9q=on}
      mask prompts: p2_3q "Power and Voltage Ratings [MVA, kV]"; p4_5q "Active and Reactive Powers [p.u.  p.u.]"; p6_7q "Maximum and Minimum Allowable Voltage [p.u.   p.u.]"; p8q "Allow conversion to impendance for min or max voltage"; p9q "Connected"
      mask help:
      | This block defines a constant power load:
      |
      | P = Pcost.
      | Q = Qcost.
      mask CallbackString: |||fm_block|fm_block
      mask Display: plot([1 -0.5 -0.5 1],[0 0.866 -0.866 0])
  PQ69 : PMComponent  Tag=PSATblock  Description=Power Flow  PhysicalDomain=psatdomain  LeftPortType=p1  RightPortType=p1  LConnTagsString=__newl0  mask(PQ){p2_3q=[100 230], p4_5q=[1.0215*0.25 0.4947*0.25]*1.0722, p6_7q=[1.2  0.8], p8q=off, p9q=on}
      mask prompts: p2_3q "Power and Voltage Ratings [MVA, kV]"; p4_5q "Active and Reactive Powers [p.u.  p.u.]"; p6_7q "Maximum and Minimum Allowable Voltage [p.u.   p.u.]"; p8q "Allow conversion to impendance for min or max voltage"; p9q "Connected"
      mask help:
      | This block defines a constant power load:
      |
      | P = Pcost.
      | Q = Qcost.
      mask CallbackString: |||fm_block|fm_block
      mask Display: plot([1 -0.5 -0.5 1],[0 0.866 -0.866 0])
  PQ7 : PMComponent  Tag=PSATblock  Description=Power Flow  PhysicalDomain=psatdomain  LeftPortType=p1  RightPortType=p1  LConnTagsString=__newl0  mask(PQ){p2_3q=[100  230], p4_5q=[3.4447 1.6955]*1.0722, p6_7q=[1.2  0.8], p8q=off, p9q=on}
      mask prompts: p2_3q "Power and Voltage Ratings [MVA, kV]"; p4_5q "Active and Reactive Powers [p.u.  p.u.]"; p6_7q "Maximum and Minimum Allowable Voltage [p.u.   p.u.]"; p8q "Allow conversion to impendance for min or max voltage"; p9q "Connected"
      mask help:
      | This block defines a constant power load:
      |
      | P = Pcost.
      | Q = Qcost.
      mask CallbackString: |||fm_block|fm_block
      mask Display: plot([1 -0.5 -0.5 1],[0 0.866 -0.866 0])
  PQ70 : PMComponent  Tag=PSATblock  Description=Power Flow  PhysicalDomain=psatdomain  LeftPortType=p1  RightPortType=p1  LConnTagsString=__newl0  mask(PQ){p2_3q=[100 115], p4_5q=[1.0215*0.25 0.4947*0.25]*1.0722, p6_7q=[1.2  0.8], p8q=off, p9q=on}
      mask prompts: p2_3q "Power and Voltage Ratings [MVA, kV]"; p4_5q "Active and Reactive Powers [p.u.  p.u.]"; p6_7q "Maximum and Minimum Allowable Voltage [p.u.   p.u.]"; p8q "Allow conversion to impendance for min or max voltage"; p9q "Connected"
      mask help:
      | This block defines a constant power load:
      |
      | P = Pcost.
      | Q = Qcost.
      mask CallbackString: |||fm_block|fm_block
      mask Display: plot([1 -0.5 -0.5 1],[0 0.866 -0.866 0])
  PQ71 : PMComponent  Tag=PSATblock  Description=Power Flow  PhysicalDomain=psatdomain  LeftPortType=p1  RightPortType=p1  LConnTagsString=__newl0  mask(PQ){p2_3q=[100 115], p4_5q=[1.0215*0.25 0.4947*0.25]*1.0722, p6_7q=[1.2  0.8], p8q=off, p9q=on}
      mask prompts: p2_3q "Power and Voltage Ratings [MVA, kV]"; p4_5q "Active and Reactive Powers [p.u.  p.u.]"; p6_7q "Maximum and Minimum Allowable Voltage [p.u.   p.u.]"; p8q "Allow conversion to impendance for min or max voltage"; p9q "Connected"
      mask help:
      | This block defines a constant power load:
      |
      | P = Pcost.
      | Q = Qcost.
      mask CallbackString: |||fm_block|fm_block
      mask Display: plot([1 -0.5 -0.5 1],[0 0.866 -0.866 0])
  PQ72 : PMComponent  Tag=PSATblock  Description=Power Flow  PhysicalDomain=psatdomain  LeftPortType=p1  RightPortType=p1  LConnTagsString=__newl0  mask(PQ){p2_3q=[100 115], p4_5q=[1.5322*0.1 0.7421*0.1]*1.0722, p6_7q=[1.2  0.8], p8q=off, p9q=on}
      mask prompts: p2_3q "Power and Voltage Ratings [MVA, kV]"; p4_5q "Active and Reactive Powers [p.u.  p.u.]"; p6_7q "Maximum and Minimum Allowable Voltage [p.u.   p.u.]"; p8q "Allow conversion to impendance for min or max voltage"; p9q "Connected"
      mask help:
      | This block defines a constant power load:
      |
      | P = Pcost.
      | Q = Qcost.
      mask CallbackString: |||fm_block|fm_block
      mask Display: plot([1 -0.5 -0.5 1],[0 0.866 -0.866 0])
  PQ73 : PMComponent  Tag=PSATblock  Description=Power Flow  PhysicalDomain=psatdomain  LeftPortType=p1  RightPortType=p1  LConnTagsString=__newl0  mask(PQ){p2_3q=[100 115], p4_5q=[1.5322*0.6 0.7421*0.6]*1.0722, p6_7q=[1.2  0.8], p8q=off, p9q=on}
      mask prompts: p2_3q "Power and Voltage Ratings [MVA, kV]"; p4_5q "Active and Reactive Powers [p.u.  p.u.]"; p6_7q "Maximum and Minimum Allowable Voltage [p.u.   p.u.]"; p8q "Allow conversion to impendance for min or max voltage"; p9q "Connected"
      mask help:
      | This block defines a constant power load:
      |
      | P = Pcost.
      | Q = Qcost.
      mask CallbackString: |||fm_block|fm_block
      mask Display: plot([1 -0.5 -0.5 1],[0 0.866 -0.866 0])
  PQ8 : PMComponent  Tag=PSATblock  Description=Power Flow  PhysicalDomain=psatdomain  LeftPortType=p1  RightPortType=p1  LConnTagsString=__newl0  mask(PQ){p2_3q=[100  230], p4_5q=[0.4865 0.2356]*1.0722, p6_7q=[1.2  0.8], p8q=off, p9q=on}
      mask prompts: p2_3q "Power and Voltage Ratings [MVA, kV]"; p4_5q "Active and Reactive Powers [p.u.  p.u.]"; p6_7q "Maximum and Minimum Allowable Voltage [p.u.   p.u.]"; p8q "Allow conversion to impendance for min or max voltage"; p9q "Connected"
      mask help:
      | This block defines a constant power load:
      |
      | P = Pcost.
      | Q = Qcost.
      mask CallbackString: |||fm_block|fm_block
      mask Display: plot([1 -0.5 -0.5 1],[0 0.866 -0.866 0])
  PQ9 : PMComponent  Tag=PSATblock  Description=Power Flow  PhysicalDomain=psatdomain  LeftPortType=p1  RightPortType=p1  LConnTagsString=__newl0  mask(PQ){p2_3q=[100 230], p4_5q=[0.8695 0.6170]*1.0722, p6_7q=[1.2  0.8], p8q=off, p9q=on}
      mask prompts: p2_3q "Power and Voltage Ratings [MVA, kV]"; p4_5q "Active and Reactive Powers [p.u.  p.u.]"; p6_7q "Maximum and Minimum Allowable Voltage [p.u.   p.u.]"; p8q "Allow conversion to impendance for min or max voltage"; p9q "Connected"
      mask help:
      | This block defines a constant power load:
      |
      | P = Pcost.
      | Q = Qcost.
      mask CallbackString: |||fm_block|fm_block
      mask Display: plot([1 -0.5 -0.5 1],[0 0.866 -0.866 0])
  PV : PMComponent  Tag=PSATblock  Description=Power Flow  PhysicalDomain=psatdomain  LeftPortType=p1  RightPortType=p1  RConnTagsString=__newr0  mask(PV){p2_3q=[100  115], p4q=2.6539+1.75, p5q=1.05, p6_7q=[0.8  -0.2], p8_9q=[1.1  0.9], p10q=1, p11q=on}
      mask prompts: p2_3q "Power and Voltage Ratings [MVA, kV]"; p4q "Active Power [p.u.]"; p5q "Voltage Magnitude [p.u.]"; p6_7q "Qmax and Qmin [p.u.  p.u.]"; p8_9q "Vmax and Vmin [p.u.  p.u.]"; p10q "Loss Participation Factor"; p11q "Connected"
      mask help:
      | This block defines a PV bus for load flow studies:
      |
      | P = Pcost.
      | V = Vdes.
      mask init:
      | [x,y] = fm_draw('circle');
      | [xp,yp] = fm_draw('P');
      mask CallbackString: ||||||fm_block
      mask Display:
      | plot(x,y)
      | color('blue')
      | plot(0.3*xp-0.35,0.6*yp,[0.1 0.3 0.5],[0.3 -0.3 0.3])
  PV1 : PMComponent  Tag=PSATblock  Description=Power Flow  PhysicalDomain=psatdomain  LeftPortType=p1  RightPortType=p1  RConnTagsString=__newr0  mask(PV){p2_3q=[100  115], p4q=5.6441*0.5, p5q=1.04, p6_7q=[0.8  -0.2], p8_9q=[1.1  0.9], p10q=1, p11q=on}
      mask prompts: p2_3q "Power and Voltage Ratings [MVA, kV]"; p4q "Active Power [p.u.]"; p5q "Voltage Magnitude [p.u.]"; p6_7q "Qmax and Qmin [p.u.  p.u.]"; p8_9q "Vmax and Vmin [p.u.  p.u.]"; p10q "Loss Participation Factor"; p11q "Connected"
      mask help:
      | This block defines a PV bus for load flow studies:
      |
      | P = Pcost.
      | V = Vdes.
      mask init:
      | [x,y] = fm_draw('circle');
      | [xp,yp] = fm_draw('P');
      mask CallbackString: ||||||fm_block
      mask Display:
      | plot(x,y)
      | color('blue')
      | plot(0.3*xp-0.35,0.6*yp,[0.1 0.3 0.5],[0.3 -0.3 0.3])
  PV10 : PMComponent  Tag=PSATblock  Description=Power Flow  PhysicalDomain=psatdomain  LeftPortType=p1  RightPortType=p1  RConnTagsString=__newr0  mask(PV){p2_3q=[100  138], p4q=10.4361, p5q=1.05, p6_7q=[0.8  -0.2], p8_9q=[1.1  0.9], p10q=1, p11q=on}
      mask prompts: p2_3q "Power and Voltage Ratings [MVA, kV]"; p4q "Active Power [p.u.]"; p5q "Voltage Magnitude [p.u.]"; p6_7q "Qmax and Qmin [p.u.  p.u.]"; p8_9q "Vmax and Vmin [p.u.  p.u.]"; p10q "Loss Participation Factor"; p11q "Connected"
      mask help:
      | This block defines a PV bus for load flow studies:
      |
      | P = Pcost.
      | V = Vdes.
      mask init:
      | [x,y] = fm_draw('circle');
      | [xp,yp] = fm_draw('P');
      mask CallbackString: ||||||fm_block
      mask Display:
      | plot(x,y)
      | color('blue')
      | plot(0.3*xp-0.35,0.6*yp,[0.1 0.3 0.5],[0.3 -0.3 0.3])
  PV11 : PMComponent  Tag=PSATblock  Description=Power Flow  PhysicalDomain=psatdomain  LeftPortType=p1  RightPortType=p1  RConnTagsString=__newr0  mask(PV){p2_3q=[100  400], p4q=13.1628, p5q=1.03, p6_7q=[0.8  -0.2], p8_9q=[1.1  0.9], p10q=1, p11q=on}
      mask prompts: p2_3q "Power and Voltage Ratings [MVA, kV]"; p4q "Active Power [p.u.]"; p5q "Voltage Magnitude [p.u.]"; p6_7q "Qmax and Qmin [p.u.  p.u.]"; p8_9q "Vmax and Vmin [p.u.  p.u.]"; p10q "Loss Participation Factor"; p11q "Connected"
      mask help:
      | This block defines a PV bus for load flow studies:
      |
      | P = Pcost.
      | V = Vdes.
      mask init:
      | [x,y] = fm_draw('circle');
      | [xp,yp] = fm_draw('P');
      mask CallbackString: ||||||fm_block
      mask Display:
      | plot(x,y)
      | color('blue')
      | plot(0.3*xp-0.35,0.6*yp,[0.1 0.3 0.5],[0.3 -0.3 0.3])
  PV12 : PMComponent  Tag=PSATblock  Description=Power Flow  PhysicalDomain=psatdomain  LeftPortType=p1  RightPortType=p1  RConnTagsString=__newr0  mask(PV){p2_3q=[100  230], p4q=2.9239, p5q=1.03, p6_7q=[0.8  -0.2], p8_9q=[1.1  0.9], p10q=1, p11q=on}
      mask prompts: p2_3q "Power and Voltage Ratings [MVA, kV]"; p4q "Active Power [p.u.]"; p5q "Voltage Magnitude [p.u.]"; p6_7q "Qmax and Qmin [p.u.  p.u.]"; p8_9q "Vmax and Vmin [p.u.  p.u.]"; p10q "Loss Participation Factor"; p11q "Connected"
      mask help:
      | This block defines a PV bus for load flow studies:
      |
      | P = Pcost.
      | V = Vdes.
      mask init:
      | [x,y] = fm_draw('circle');
      | [xp,yp] = fm_draw('P');
      mask CallbackString: ||||||fm_block
      mask Display:
      | plot(x,y)
      | color('blue')
      | plot(0.3*xp-0.35,0.6*yp,[0.1 0.3 0.5],[0.3 -0.3 0.3])
  PV13 : PMComponent  Tag=PSATblock  Description=Power Flow  PhysicalDomain=psatdomain  LeftPortType=p1  RightPortType=p1  RConnTagsString=__newr0  mask(PV){p2_3q=[100  230], p4q=2.1010+2.8, p5q=1.05, p6_7q=[0.8  -0.2], p8_9q=[1.1  0.9], p10q=1, p11q=on}
      mask prompts: p2_3q "Power and Voltage Ratings [MVA, kV]"; p4q "Active Power [p.u.]"; p5q "Voltage Magnitude [p.u.]"; p6_7q "Qmax and Qmin [p.u.  p.u.]"; p8_9q "Vmax and Vmin [p.u.  p.u.]"; p10q "Loss Participation Factor"; p11q "Connected"
      mask help:
      | This block defines a PV bus for load flow studies:
      |
      | P = Pcost.
      | V = Vdes.
      mask init:
      | [x,y] = fm_draw('circle');
      | [xp,yp] = fm_draw('P');
      mask CallbackString: ||||||fm_block
      mask Display:
      | plot(x,y)
      | color('blue')
      | plot(0.3*xp-0.35,0.6*yp,[0.1 0.3 0.5],[0.3 -0.3 0.3])
  PV14 : PMComponent  Tag=PSATblock  Description=Power Flow  PhysicalDomain=psatdomain  LeftPortType=p1  RightPortType=p1  RConnTagsString=__newr0  mask(PV){p2_3q=[100  400], p4q=14.6386, p5q=1.03, p6_7q=[0.8  -0.2], p8_9q=[1.1  0.9], p10q=1, p11q=on}
      mask prompts: p2_3q "Power and Voltage Ratings [MVA, kV]"; p4q "Active Power [p.u.]"; p5q "Voltage Magnitude [p.u.]"; p6_7q "Qmax and Qmin [p.u.  p.u.]"; p8_9q "Vmax and Vmin [p.u.  p.u.]"; p10q "Loss Participation Factor"; p11q "Connected"
      mask help:
      | This block defines a PV bus for load flow studies:
      |
      | P = Pcost.
      | V = Vdes.
      mask init:
      | [x,y] = fm_draw('circle');
      | [xp,yp] = fm_draw('P');
      mask CallbackString: ||||||fm_block
      mask Display:
      | plot(x,y)
      | color('blue')
      | plot(0.3*xp-0.35,0.6*yp,[0.1 0.3 0.5],[0.3 -0.3 0.3])
  PV15 : PMComponent  Tag=PSATblock  Description=Power Flow  PhysicalDomain=psatdomain  LeftPortType=p1  RightPortType=p1  RConnTagsString=__newr0  mask(PV){p2_3q=[100  230], p4q=5.04, p5q=1.02, p6_7q=[0.8  -0.2], p8_9q=[1.1  0.9], p10q=1, p11q=on}
      mask prompts: p2_3q "Power and Voltage Ratings [MVA, kV]"; p4q "Active Power [p.u.]"; p5q "Voltage Magnitude [p.u.]"; p6_7q "Qmax and Qmin [p.u.  p.u.]"; p8_9q "Vmax and Vmin [p.u.  p.u.]"; p10q "Loss Participation Factor"; p11q "Connected"
      mask help:
      | This block defines a PV bus for load flow studies:
      |
      | P = Pcost.
      | V = Vdes.
      mask init:
      | [x,y] = fm_draw('circle');
      | [xp,yp] = fm_draw('P');
      mask CallbackString: ||||||fm_block
      mask Display:
      | plot(x,y)
      | color('blue')
      | plot(0.3*xp-0.35,0.6*yp,[0.1 0.3 0.5],[0.3 -0.3 0.3])
  PV16 : PMComponent  Tag=PSATblock  Description=Power Flow  PhysicalDomain=psatdomain  LeftPortType=p1  RightPortType=p1  RConnTagsString=__newr0  mask(PV){p2_3q=[100  400], p4q=4.2*0.5, p5q=1.02, p6_7q=[0.8  -0.2], p8_9q=[1.1  0.9], p10q=1, p11q=on}
      mask prompts: p2_3q "Power and Voltage Ratings [MVA, kV]"; p4q "Active Power [p.u.]"; p5q "Voltage Magnitude [p.u.]"; p6_7q "Qmax and Qmin [p.u.  p.u.]"; p8_9q "Vmax and Vmin [p.u.  p.u.]"; p10q "Loss Participation Factor"; p11q "Connected"
      mask help:
      | This block defines a PV bus for load flow studies:
      |
      | P = Pcost.
      | V = Vdes.
      mask init:
      | [x,y] = fm_draw('circle');
      | [xp,yp] = fm_draw('P');
      mask CallbackString: ||||||fm_block
      mask Display:
      | plot(x,y)
      | color('blue')
      | plot(0.3*xp-0.35,0.6*yp,[0.1 0.3 0.5],[0.3 -0.3 0.3])
  PV17 : PMComponent  Tag=PSATblock  Description=Power Flow  PhysicalDomain=psatdomain  LeftPortType=p1  RightPortType=p1  RConnTagsString=__newr0  mask(PV){p2_3q=[100  400], p4q=4.2*0.5, p5q=1.02, p6_7q=[0.8  -0.2], p8_9q=[1.1  0.9], p10q=1, p11q=on}
      mask prompts: p2_3q "Power and Voltage Ratings [MVA, kV]"; p4q "Active Power [p.u.]"; p5q "Voltage Magnitude [p.u.]"; p6_7q "Qmax and Qmin [p.u.  p.u.]"; p8_9q "Vmax and Vmin [p.u.  p.u.]"; p10q "Loss Participation Factor"; p11q "Connected"
      mask help:
      | This block defines a PV bus for load flow studies:
      |
      | P = Pcost.
      | V = Vdes.
      mask init:
      | [x,y] = fm_draw('circle');
      | [xp,yp] = fm_draw('P');
      mask CallbackString: ||||||fm_block
      mask Display:
      | plot(x,y)
      | color('blue')
      | plot(0.3*xp-0.35,0.6*yp,[0.1 0.3 0.5],[0.3 -0.3 0.3])
  PV18 : PMComponent  Tag=PSATblock  Description=Power Flow  PhysicalDomain=psatdomain  LeftPortType=p1  RightPortType=p1  RConnTagsString=__newr0  mask(PV){p2_3q=[100  230], p4q=1.05, p5q=1.02, p6_7q=[0.8  -0.2], p8_9q=[1.1  0.9], p10q=1, p11q=on}
      mask prompts: p2_3q "Power and Voltage Ratings [MVA, kV]"; p4q "Active Power [p.u.]"; p5q "Voltage Magnitude [p.u.]"; p6_7q "Qmax and Qmin [p.u.  p.u.]"; p8_9q "Vmax and Vmin [p.u.  p.u.]"; p10q "Loss Participation Factor"; p11q "Connected"
      mask help:
      | This block defines a PV bus for load flow studies:
      |
      | P = Pcost.
      | V = Vdes.
      mask init:
      | [x,y] = fm_draw('circle');
      | [xp,yp] = fm_draw('P');
      mask CallbackString: ||||||fm_block
      mask Display:
      | plot(x,y)
      | color('blue')
      | plot(0.3*xp-0.35,0.6*yp,[0.1 0.3 0.5],[0.3 -0.3 0.3])
  PV19 : PMComponent  Tag=PSATblock  Description=Power Flow  PhysicalDomain=psatdomain  LeftPortType=p1  RightPortType=p1  RConnTagsString=__newr0  mask(PV){p2_3q=[100  230], p4q=2.997, p5q=1.02, p6_7q=[0.8  -0.2], p8_9q=[1.1  0.9], p10q=1, p11q=on}
      mask prompts: p2_3q "Power and Voltage Ratings [MVA, kV]"; p4q "Active Power [p.u.]"; p5q "Voltage Magnitude [p.u.]"; p6_7q "Qmax and Qmin [p.u.  p.u.]"; p8_9q "Vmax and Vmin [p.u.  p.u.]"; p10q "Loss Participation Factor"; p11q "Connected"
      mask help:
      | This block defines a PV bus for load flow studies:
      |
      | P = Pcost.
      | V = Vdes.
      mask init:
      | [x,y] = fm_draw('circle');
      | [xp,yp] = fm_draw('P');
      mask CallbackString: ||||||fm_block
      mask Display:
      | plot(x,y)
      | color('blue')
      | plot(0.3*xp-0.35,0.6*yp,[0.1 0.3 0.5],[0.3 -0.3 0.3])
  PV2 : PMComponent  Tag=PSATblock  Description=Power Flow  PhysicalDomain=psatdomain  LeftPortType=p1  RightPortType=p1  RConnTagsString=__newr0  mask(PV){p2_3q=[100  230], p4q=11.1020, p5q=1.05, p6_7q=[0.8  -0.2], p8_9q=[1.1  0.9], p10q=1, p11q=on}
      mask prompts: p2_3q "Power and Voltage Ratings [MVA, kV]"; p4q "Active Power [p.u.]"; p5q "Voltage Magnitude [p.u.]"; p6_7q "Qmax and Qmin [p.u.  p.u.]"; p8_9q "Vmax and Vmin [p.u.  p.u.]"; p10q "Loss Participation Factor"; p11q "Connected"
      mask help:
      | This block defines a PV bus for load flow studies:
      |
      | P = Pcost.
      | V = Vdes.
      mask init:
      | [x,y] = fm_draw('circle');
      | [xp,yp] = fm_draw('P');
      mask CallbackString: ||||||fm_block
      mask Display:
      | plot(x,y)
      | color('blue')
      | plot(0.3*xp-0.35,0.6*yp,[0.1 0.3 0.5],[0.3 -0.3 0.3])
  PV20 : PMComponent  Tag=PSATblock  Description=Power Flow  PhysicalDomain=psatdomain  LeftPortType=p1  RightPortType=p1  RConnTagsString=__newr0  mask(PV){p2_3q=[100  230], p4q=7.77, p5q=1.02, p6_7q=[0.8  -0.2], p8_9q=[1.1  0.9], p10q=1, p11q=on}
      mask prompts: p2_3q "Power and Voltage Ratings [MVA, kV]"; p4q "Active Power [p.u.]"; p5q "Voltage Magnitude [p.u.]"; p6_7q "Qmax and Qmin [p.u.  p.u.]"; p8_9q "Vmax and Vmin [p.u.  p.u.]"; p10q "Loss Participation Factor"; p11q "Connected"
      mask help:
      | This block defines a PV bus for load flow studies:
      |
      | P = Pcost.
      | V = Vdes.
      mask init:
      | [x,y] = fm_draw('circle');
      | [xp,yp] = fm_draw('P');
      mask CallbackString: ||||||fm_block
      mask Display:
      | plot(x,y)
      | color('blue')
      | plot(0.3*xp-0.35,0.6*yp,[0.1 0.3 0.5],[0.3 -0.3 0.3])
  PV22 : PMComponent  Tag=PSATblock  Description=Power Flow  PhysicalDomain=psatdomain  LeftPortType=p1  RightPortType=p1  RConnTagsString=__newr0  mask(PV){p2_3q=[100  230], p4q=1.1667, p5q=1.05, p6_7q=[0.8  -0.2], p8_9q=[1.1  0.9], p10q=1, p11q=on}
      mask prompts: p2_3q "Power and Voltage Ratings [MVA, kV]"; p4q "Active Power [p.u.]"; p5q "Voltage Magnitude [p.u.]"; p6_7q "Qmax and Qmin [p.u.  p.u.]"; p8_9q "Vmax and Vmin [p.u.  p.u.]"; p10q "Loss Participation Factor"; p11q "Connected"
      mask help:
      | This block defines a PV bus for load flow studies:
      |
      | P = Pcost.
      | V = Vdes.
      mask init:
      | [x,y] = fm_draw('circle');
      | [xp,yp] = fm_draw('P');
      mask CallbackString: ||||||fm_block
      mask Display:
      | plot(x,y)
      | color('blue')
      | plot(0.3*xp-0.35,0.6*yp,[0.1 0.3 0.5],[0.3 -0.3 0.3])
  PV3 : PMComponent  Tag=PSATblock  Description=Power Flow  PhysicalDomain=psatdomain  LeftPortType=p1  RightPortType=p1  RConnTagsString=__newr0  mask(PV){p2_3q=[100  230], p4q=2.8610, p5q=1.05, p6_7q=[0.8  -0.2], p8_9q=[1.1  0.9], p10q=1, p11q=on}
      mask prompts: p2_3q "Power and Voltage Ratings [MVA, kV]"; p4q "Active Power [p.u.]"; p5q "Voltage Magnitude [p.u.]"; p6_7q "Qmax and Qmin [p.u.  p.u.]"; p8_9q "Vmax and Vmin [p.u.  p.u.]"; p10q "Loss Participation Factor"; p11q "Connected"
      mask help:
      | This block defines a PV bus for load flow studies:
      |
      | P = Pcost.
      | V = Vdes.
      mask init:
      | [x,y] = fm_draw('circle');
      | [xp,yp] = fm_draw('P');
      mask CallbackString: ||||||fm_block
      mask Display:
      | plot(x,y)
      | color('blue')
      | plot(0.3*xp-0.35,0.6*yp,[0.1 0.3 0.5],[0.3 -0.3 0.3])
  PV38 : PMComponent  Tag=PSATblock  Description=Power Flow  PhysicalDomain=psatdomain  LeftPortType=p1  RightPortType=p1  RConnTagsString=__newr0  mask(PV){p2_3q=[100  115], p4q=5.6441*0.5, p5q=1.07, p6_7q=[0.8  -0.2], p8_9q=[1.1  0.9], p10q=1, p11q=on}
      mask prompts: p2_3q "Power and Voltage Ratings [MVA, kV]"; p4q "Active Power [p.u.]"; p5q "Voltage Magnitude [p.u.]"; p6_7q "Qmax and Qmin [p.u.  p.u.]"; p8_9q "Vmax and Vmin [p.u.  p.u.]"; p10q "Loss Participation Factor"; p11q "Connected"
      mask help:
      | This block defines a PV bus for load flow studies:
      |
      | P = Pcost.
      | V = Vdes.
      mask init:
      | [x,y] = fm_draw('circle');
      | [xp,yp] = fm_draw('P');
      mask CallbackString: ||||||fm_block
      mask Display:
      | plot(x,y)
      | color('blue')
      | plot(0.3*xp-0.35,0.6*yp,[0.1 0.3 0.5],[0.3 -0.3 0.3])
  PV4 : PMComponent  Tag=PSATblock  Description=Power Flow  PhysicalDomain=psatdomain  LeftPortType=p1  RightPortType=p1  RConnTagsString=__newr0  mask(PV){p2_3q=[100  230], p4q=1.7982, p5q=1.05, p6_7q=[0.8  -0.2], p8_9q=[1.1  0.9], p10q=1, p11q=on}
      mask prompts: p2_3q "Power and Voltage Ratings [MVA, kV]"; p4q "Active Power [p.u.]"; p5q "Voltage Magnitude [p.u.]"; p6_7q "Qmax and Qmin [p.u.  p.u.]"; p8_9q "Vmax and Vmin [p.u.  p.u.]"; p10q "Loss Participation Factor"; p11q "Connected"
      mask help:
      | This block defines a PV bus for load flow studies:
      |
      | P = Pcost.
      | V = Vdes.
      mask init:
      | [x,y] = fm_draw('circle');
      | [xp,yp] = fm_draw('P');
      mask CallbackString: ||||||fm_block
      mask Display:
      | plot(x,y)
      | color('blue')
      | plot(0.3*xp-0.35,0.6*yp,[0.1 0.3 0.5],[0.3 -0.3 0.3])
  PV5 : PMComponent  Tag=PSATblock  Description=Power Flow  PhysicalDomain=psatdomain  LeftPortType=p1  RightPortType=p1  RConnTagsString=__newr0  mask(PV){p2_3q=[100  138], p4q=4.62, p5q=1.05, p6_7q=[0.8  -0.2], p8_9q=[1.1  0.9], p10q=1, p11q=on}
      mask prompts: p2_3q "Power and Voltage Ratings [MVA, kV]"; p4q "Active Power [p.u.]"; p5q "Voltage Magnitude [p.u.]"; p6_7q "Qmax and Qmin [p.u.  p.u.]"; p8_9q "Vmax and Vmin [p.u.  p.u.]"; p10q "Loss Participation Factor"; p11q "Connected"
      mask help:
      | This block defines a PV bus for load flow studies:
      |
      | P = Pcost.
      | V = Vdes.
      mask init:
      | [x,y] = fm_draw('circle');
      | [xp,yp] = fm_draw('P');
      mask CallbackString: ||||||fm_block
      mask Display:
      | plot(x,y)
      | color('blue')
      | plot(0.3*xp-0.35,0.6*yp,[0.1 0.3 0.5],[0.3 -0.3 0.3])
  PV6 : PMComponent  Tag=PSATblock  Description=Power Flow  PhysicalDomain=psatdomain  LeftPortType=p1  RightPortType=p1  RConnTagsString=__newr0  mask(PV){p2_3q=[100  230], p4q=2.6539+4.83, p5q=1.02, p6_7q=[0.8  -0.2], p8_9q=[1.1  0.9], p10q=1, p11q=on}
      mask prompts: p2_3q "Power and Voltage Ratings [MVA, kV]"; p4q "Active Power [p.u.]"; p5q "Voltage Magnitude [p.u.]"; p6_7q "Qmax and Qmin [p.u.  p.u.]"; p8_9q "Vmax and Vmin [p.u.  p.u.]"; p10q "Loss Participation Factor"; p11q "Connected"
      mask help:
      | This block defines a PV bus for load flow studies:
      |
      | P = Pcost.
      | V = Vdes.
      mask init:
      | [x,y] = fm_draw('circle');
      | [xp,yp] = fm_draw('P');
      mask CallbackString: ||||||fm_block
      mask Display:
      | plot(x,y)
      | color('blue')
      | plot(0.3*xp-0.35,0.6*yp,[0.1 0.3 0.5],[0.3 -0.3 0.3])
  PV7 : PMComponent  Tag=PSATblock  Description=Power Flow  PhysicalDomain=psatdomain  LeftPortType=p1  RightPortType=p1  RConnTagsString=__newr0  mask(PV){p2_3q=[100  400], p4q=11.7691, p5q=1.05, p6_7q=[0.8  -0.2], p8_9q=[1.1  0.9], p10q=1, p11q=on}
      mask prompts: p2_3q "Power and Voltage Ratings [MVA, kV]"; p4q "Active Power [p.u.]"; p5q "Voltage Magnitude [p.u.]"; p6_7q "Qmax and Qmin [p.u.  p.u.]"; p8_9q "Vmax and Vmin [p.u.  p.u.]"; p10q "Loss Participation Factor"; p11q "Connected"
      mask help:
      | This block defines a PV bus for load flow studies:
      |
      | P = Pcost.
      | V = Vdes.
      mask init:
      | [x,y] = fm_draw('circle');
      | [xp,yp] = fm_draw('P');
      mask CallbackString: ||||||fm_block
      mask Display:
      | plot(x,y)
      | color('blue')
      | plot(0.3*xp-0.35,0.6*yp,[0.1 0.3 0.5],[0.3 -0.3 0.3])
  PV8 : PMComponent  Tag=PSATblock  Description=Power Flow  PhysicalDomain=psatdomain  LeftPortType=p1  RightPortType=p1  RConnTagsString=__newr0  mask(PV){p2_3q=[100  230], p4q=3.2368, p5q=1.05, p6_7q=[0.8  -0.2], p8_9q=[1.1  0.9], p10q=1, p11q=on}
      mask prompts: p2_3q "Power and Voltage Ratings [MVA, kV]"; p4q "Active Power [p.u.]"; p5q "Voltage Magnitude [p.u.]"; p6_7q "Qmax and Qmin [p.u.  p.u.]"; p8_9q "Vmax and Vmin [p.u.  p.u.]"; p10q "Loss Participation Factor"; p11q "Connected"
      mask help:
      | This block defines a PV bus for load flow studies:
      |
      | P = Pcost.
      | V = Vdes.
      mask init:
      | [x,y] = fm_draw('circle');
      | [xp,yp] = fm_draw('P');
      mask CallbackString: ||||||fm_block
      mask Display:
      | plot(x,y)
      | color('blue')
      | plot(0.3*xp-0.35,0.6*yp,[0.1 0.3 0.5],[0.3 -0.3 0.3])
  PV9 : PMComponent  Tag=PSATblock  Description=Power Flow  PhysicalDomain=psatdomain  LeftPortType=p1  RightPortType=p1  RConnTagsString=__newr0  mask(PV){p2_3q=[100  400], p4q=13.5944, p5q=1.05, p6_7q=[0.8  -0.2], p8_9q=[1.1  0.9], p10q=1, p11q=on}
      mask prompts: p2_3q "Power and Voltage Ratings [MVA, kV]"; p4q "Active Power [p.u.]"; p5q "Voltage Magnitude [p.u.]"; p6_7q "Qmax and Qmin [p.u.  p.u.]"; p8_9q "Vmax and Vmin [p.u.  p.u.]"; p10q "Loss Participation Factor"; p11q "Connected"
      mask help:
      | This block defines a PV bus for load flow studies:
      |
      | P = Pcost.
      | V = Vdes.
      mask init:
      | [x,y] = fm_draw('circle');
      | [xp,yp] = fm_draw('P');
      mask CallbackString: ||||||fm_block
      mask Display:
      | plot(x,y)
      | color('blue')
      | plot(0.3*xp-0.35,0.6*yp,[0.1 0.3 0.5],[0.3 -0.3 0.3])
  Palital 400kV : PMComponent  Tag=PSATblock  Description=Connection  PhysicalDomain=psatdomain  LeftPortType=p1  RightPortType=p1  LConnTagsString=__newl0|__newl1|__newl2  RConnTagsString=__newr0|__newr1  mask(Bus){in=3, out=2, p2q=400, p3_4q=[1.0189    -0.15846], p5q=1, p6q=1}
      mask prompts: in "Number of inputs:"; out "Number of outputs:"; p2q "Voltage Rating [kV]"; p3_4q "Voltage initial guess [p.u.  rad]"; p5q "Area number"; p6q "Region number"
      mask help: Bus block.
      mask init:
      | fm_inout
      settings: AttributesFormatString="|V| =  0.9789 p.u.\\n<V  = -0.1293 rad"
      mask CallbackString: ||||fm_block|
      mask Display: plot([0 1 1 0 0],[0 0 1 1 0])
  Papelon 230kV : PMComponent  Tag=PSATblock  Description=Connection  PhysicalDomain=psatdomain  LeftPortType=p1  RightPortType=p1  LConnTagsString=__newl0|__newl1  RConnTagsString=__newr0|__newr1|__newr2  mask(Bus){in=2, out=3, p2q=230, p3_4q=[0.99933     -0.4575], p5q=1, p6q=1}
      mask prompts: in "Number of inputs:"; out "Number of outputs:"; p2q "Voltage Rating [kV]"; p3_4q "Voltage initial guess [p.u.  rad]"; p5q "Area number"; p6q "Region number"
      mask help: Bus block.
      mask init:
      | fm_inout
      settings: AttributesFormatString="|V| =  1.0197 p.u.\\n<V  = -0.2857 rad"
      mask CallbackString: ||||fm_block|
      mask Display: plot([0 1 1 0 0],[0 0 1 1 0])
  Peonias : PMComponent  Tag=PSATblock  Description=Connection  PhysicalDomain=psatdomain  LeftPortType=p1  RightPortType=p1  LConnTagsString=__newl0|__newl1  RConnTagsString=__newr0|__newr1  mask(Bus){in=2, out=2, p2q=230, p3_4q=[0.98842    -0.82663], p5q=1, p6q=1}
      mask prompts: in "Number of inputs:"; out "Number of outputs:"; p2q "Voltage Rating [kV]"; p3_4q "Voltage initial guess [p.u.  rad]"; p5q "Area number"; p6q "Region number"
      mask help: Bus block.
      mask init:
      | fm_inout
      settings: AttributesFormatString="|V| =  1.0343 p.u.\\n<V  = -0.3763 rad"
      mask CallbackString: ||||fm_block|
      mask Display: plot([0 1 1 0 0],[0 0 1 1 0])
  Planta Centro 230kV : PMComponent  Tag=PSATblock  Description=Connection  PhysicalDomain=psatdomain  LeftPortType=p1  RightPortType=p1  LConnTagsString=__newl0|__newl1  RConnTagsString=__newr0|__newr1|__newr2|__newr3|__newr4|__newr5  mask(Bus){in=2, out=6, p2q=230, p3_4q=[0.99115    -0.50302], p5q=1, p6q=1}
      mask prompts: in "Number of inputs:"; out "Number of outputs:"; p2q "Voltage Rating [kV]"; p3_4q "Voltage initial guess [p.u.  rad]"; p5q "Area number"; p6q "Region number"
      mask help: Bus block.
      mask init:
      | fm_inout
      settings: AttributesFormatString="|V| =  0.983  p.u.\\n<V  = -0.2708 rad"
      mask CallbackString: ||||fm_block|
      mask Display: plot([0 1 1 0 0],[0 0 1 1 0])
  Planta Centro 400kV : PMComponent  Tag=PSATblock  Description=Connection  PhysicalDomain=psatdomain  LeftPortType=p1  RightPortType=p1  LConnTagsString=__newl0|__newl1|__newl2  RConnTagsString=__newr0|__newr1|__newr2|__newr3  mask(Bus){in=3, out=4, p2q=400, p3_4q=[1.05    -0.41469], p5q=1, p6q=1}
      mask prompts: in "Number of inputs:"; out "Number of outputs:"; p2q "Voltage Rating [kV]"; p3_4q "Voltage initial guess [p.u.  rad]"; p5q "Area number"; p6q "Region number"
      mask help: Bus block.
      mask init:
      | fm_inout
      settings: AttributesFormatString="|V| =  1.05   p.u.\\n<V  = -0.1935 rad"
      mask CallbackString: ||||fm_block|
      mask Display: plot([0 1 1 0 0],[0 0 1 1 0])
  Planta Paez 230kV : PMComponent  Tag=PSATblock  Description=Connection  PhysicalDomain=psatdomain  LeftPortType=p1  RightPortType=p1  LConnTagsString=__newl0|__newl1|__newl2  RConnTagsString=__newr0|__newr1|__newr2  mask(Bus){in=3, out=3, p2q=230, p3_4q=[1.07    -0.62878], p5q=1, p6q=1}
      mask prompts: in "Number of inputs:"; out "Number of outputs:"; p2q "Voltage Rating [kV]"; p3_4q "Voltage initial guess [p.u.  rad]"; p5q "Area number"; p6q "Region number"
      mask help: Bus block.
      mask init:
      | fm_inout
      settings: AttributesFormatString="|V| =  1.05   p.u.\\n<V  = -0.1964 rad"
      mask CallbackString: ||||fm_block|
      mask Display: plot([0 1 1 0 0],[0 0 1 1 0])
  Pss : Subsystem  Tag=PSATblock  Description=Controls  mask(Pss){p2q=2, p3q=omega, p4_5q=[0.05 -0.05], p6_7q=[50  0.5], p14_15q=20  5, p8_9_10_11q=[0.1 0.05 0.01 0.005], p12_13q=[25 0.5], p16_17_18_19q=[0.045  0.045  0.045  -0.045], p20_21q=[1.000  0.95], p22q=off, p23q=off}
      mask prompts: p2q "PSS model"; p3q "Input Signal"; p4_5q "Max and Min Stabilizer Output [p.u.]"; p6_7q "Gain Kw and time constant Tw  [p.u./p.u., s]"; p14_15q "Electrical power gain Kp and voltage gain Kv [p.u./p.u., p.u./p.u.]"; p8_9_10_11q "Lead-Lag time constants T1, T2, T3, T4 [s, s, s, s]"; p12_13q "Gain Ka and time constant Ta [p.u./p.u., s]"; p16_17_18_19q "Additional signal limits Va_max, Va_thr, V3_max and V3_min [p.u., p.u., p.u., p.u.]"; p20_21q "Threshold limits E_thr and w_thr [p.u., p.u.]"; p22q "Allow switch S2"; p23q "Connected"
      mask help: This block defines a Power System Stabilizer.
      mask init:
      | [xs,ys] = fm_draw('S');
      | [xp,yp] = fm_draw('P');
      mask StyleString: popup(1|2|3|4|5),popup(omega|power|voltage),edit,edit,edit,edit,edit,edit,edit,checkbox,checkbox
      mask CallbackString: fm_block||||||||||fm_block
      mask Display:
      | plot([-1.8 4.1 4.1 -1.8 -1.8],[-1.5 -1.5 1.5 1.5 -1.5])
      | color('red')
      | plot(1.5*xp-0.7,2*yp,1.2+1.5*xs,2*ys,2.8+1.5*xs,2*ys)
  Pss1 : Subsystem  Tag=PSATblock  Description=Controls  mask(Pss){p2q=2, p3q=omega, p4_5q=[10 -10], p6_7q=[50  0.5], p14_15q=20  5, p8_9_10_11q=[1.4900 2.7701e-004 1.3686 0.4544], p12_13q=[25 0.5], p16_17_18_19q=[0.045  0.045  0.045  -0.045], p20_21q=[1.000  0.95], p22q=off, p23q=off}
      mask prompts: p2q "PSS model"; p3q "Input Signal"; p4_5q "Max and Min Stabilizer Output [p.u.]"; p6_7q "Gain Kw and time constant Tw  [p.u./p.u., s]"; p14_15q "Electrical power gain Kp and voltage gain Kv [p.u./p.u., p.u./p.u.]"; p8_9_10_11q "Lead-Lag time constants T1, T2, T3, T4 [s, s, s, s]"; p12_13q "Gain Ka and time constant Ta [p.u./p.u., s]"; p16_17_18_19q "Additional signal limits Va_max, Va_thr, V3_max and V3_min [p.u., p.u., p.u., p.u.]"; p20_21q "Threshold limits E_thr and w_thr [p.u., p.u.]"; p22q "Allow switch S2"; p23q "Connected"
      mask help: This block defines a Power System Stabilizer.
      mask init:
      | [xs,ys] = fm_draw('S');
      | [xp,yp] = fm_draw('P');
      mask StyleString: popup(1|2|3|4|5),popup(omega|power|voltage),edit,edit,edit,edit,edit,edit,edit,checkbox,checkbox
      mask CallbackString: fm_block||||||||||fm_block
      mask Display:
      | plot([-1.8 4.1 4.1 -1.8 -1.8],[-1.5 -1.5 1.5 1.5 -1.5])
      | color('red')
      | plot(1.5*xp-0.7,2*yp,1.2+1.5*xs,2*ys,2.8+1.5*xs,2*ys)
  Punto Fijo I : PMComponent  Tag=PSATblock  Description=Connection  PhysicalDomain=psatdomain  LeftPortType=p1  RightPortType=p1  LConnTagsString=__newl0|__newl1  RConnTagsString=__newr0|__newr1  mask(Bus){in=2, out=2, p2q=115, p3_4q=[1.02    0.054618], p5q=1, p6q=1}
      mask prompts: in "Number of inputs:"; out "Number of outputs:"; p2q "Voltage Rating [kV]"; p3_4q "Voltage initial guess [p.u.  rad]"; p5q "Area number"; p6q "Region number"
      mask help: Bus block.
      mask init:
      | fm_inout
      settings: AttributesFormatString="|V| =  1.04   p.u.\\n<V  =  0.6831 rad"
      mask CallbackString: ||||fm_block|
      mask Display: plot([0 1 1 0 0],[0 0 1 1 0])
  Punto Fijo II : PMComponent  Tag=PSATblock  Description=Connection  PhysicalDomain=psatdomain  LeftPortType=p1  RightPortType=p1  LConnTagsString=__newl0|__newl1  RConnTagsString=__newr0|__newr1|__newr2  mask(Bus){in=2, out=3, p2q=115, p3_4q=[0.99383    0.019735], p5q=1, p6q=1}
      mask prompts: in "Number of inputs:"; out "Number of outputs:"; p2q "Voltage Rating [kV]"; p3_4q "Voltage initial guess [p.u.  rad]"; p5q "Area number"; p6q "Region number"
      mask help: Bus block.
      mask init:
      | fm_inout
      settings: AttributesFormatString="|V| =  1.0223 p.u.\\n<V  =  0.6472 rad"
      mask CallbackString: ||||fm_block|
      mask Display: plot([0 1 1 0 0],[0 0 1 1 0])
  Ramon Laguna 138kV : PMComponent  Tag=PSATblock  Description=Connection  PhysicalDomain=psatdomain  LeftPortType=p1  RightPortType=p1  LConnTagsString=__newl0|__newl1|__newl2|__newl3|__newl4  RConnTagsString=__newr0|__newr1  mask(Bus){in=5, out=2, p2q=138, p3_4q=[1.07    -0.91379], p5q=1, p6q=1}
      mask prompts: in "Number of inputs:"; out "Number of outputs:"; p2q "Voltage Rating [kV]"; p3_4q "Voltage initial guess [p.u.  rad]"; p5q "Area number"; p6q "Region number"
      mask help: Bus block.
      mask init:
      | fm_inout
      settings: AttributesFormatString="|V| =  1.05   p.u.\\n<V  = -0.3141 rad"
      mask CallbackString: ||||fm_block|
      mask Display: plot([0 1 1 0 0],[0 0 1 1 0])
  Rio Chico II : PMComponent  Tag=PSATblock  Description=Connection  PhysicalDomain=psatdomain  LeftPortType=p1  RightPortType=p1  LConnTagsString=__newl0|__newl1  RConnTagsString=__newr0  mask(Bus){in=2, out=1, p2q=230, p3_4q=[0.92904    -0.47497], p5q=1, p6q=1}
      mask prompts: in "Number of inputs:"; out "Number of outputs:"; p2q "Voltage Rating [kV]"; p3_4q "Voltage initial guess [p.u.  rad]"; p5q "Area number"; p6q "Region number"
      mask help: Bus block.
      mask init:
      | fm_inout
      settings: AttributesFormatString="|V| =  0.9774 p.u.\\n<V  = -0.2566 rad"
      mask CallbackString: ||||fm_block|
      mask Display: plot([0 1 1 0 0],[0 0 1 1 0])
  SC1 : PMComponent  Tag=PSATblock  Description=Power Flow  PhysicalDomain=psatdomain  LeftPortType=p1  RightPortType=p1  RConnTagsString=__newr0  mask(PV){p2_3q=[100  765], p5q=1.05, p6_7q=[2.8  -3], p8_9q=[1.1  0.9], p10q=1, p11q=on}
      mask prompts: p2_3q "Power and Voltage Ratings [MVA, kV]"; p5q "Voltage Magnitude [p.u.]"; p6_7q "Qmax and Qmin [p.u.  p.u.]"; p8_9q "Vmax and Vmin [p.u.  p.u.]"; p10q "Loss Participation Coefficient"; p11q "Connected"
      mask help:
      | This block defines a static synchronous compensator:
      | P = 0
      | V = Vdes
      mask init:
      | [x,y] = fm_draw('circle');
      | [xc,yc] = fm_draw('C');
      mask CallbackString: |||||fm_block
      mask Display:
      | plot(x,y,[-0.25 -0.25],[-0.25 0.25])
      | color('blue')
      | plot(0.5*xc-0.25,yc)
  SC3 : PMComponent  Tag=PSATblock  Description=Power Flow  PhysicalDomain=psatdomain  LeftPortType=p1  RightPortType=p1  RConnTagsString=__newr0  mask(PV){p2_3q=[100  765], p5q=1.05, p6_7q=[2.8  -3], p8_9q=[1.1  0.9], p10q=1, p11q=on}
      mask prompts: p2_3q "Power and Voltage Ratings [MVA, kV]"; p5q "Voltage Magnitude [p.u.]"; p6_7q "Qmax and Qmin [p.u.  p.u.]"; p8_9q "Vmax and Vmin [p.u.  p.u.]"; p10q "Loss Participation Coefficient"; p11q "Connected"
      mask help:
      | This block defines a static synchronous compensator:
      | P = 0
      | V = Vdes
      mask init:
      | [x,y] = fm_draw('circle');
      | [xc,yc] = fm_draw('C');
      mask CallbackString: |||||fm_block
      mask Display:
      | plot(x,y,[-0.25 -0.25],[-0.25 0.25])
      | color('blue')
      | plot(0.5*xc-0.25,yc)
  San Agaton : PMComponent  Tag=PSATblock  Description=Connection  PhysicalDomain=psatdomain  LeftPortType=p1  RightPortType=p1  LConnTagsString=__newl0|__newl1  RConnTagsString=__newr0|__newr1  mask(Bus){in=2, out=2, p2q=230, p3_4q=[1.07    -0.64372], p5q=1, p6q=1}
      mask prompts: in "Number of inputs:"; out "Number of outputs:"; p2q "Voltage Rating [kV]"; p3_4q "Voltage initial guess [p.u.  rad]"; p5q "Area number"; p6q "Region number"
      mask help: Bus block.
      mask init:
      | fm_inout
      settings: AttributesFormatString="|V| =  1.05   p.u.\\n<V  =  0.7082 rad"
      mask CallbackString: ||||fm_block|
      mask Display: plot([0 1 1 0 0],[0 0 1 1 0])
  San Diego 230kV : PMComponent  Tag=PSATblock  Description=Connection  PhysicalDomain=psatdomain  LeftPortType=p1  RightPortType=p1  LConnTagsString=__newl0|__newl1|__newl2|__newl3  RConnTagsString=__newr0|__newr1|__newr2  mask(Bus){in=4, out=3, p2q=230, p3_4q=[0.94718     -0.5857], p5q=1, p6q=1}
      mask prompts: in "Number of inputs:"; out "Number of outputs:"; p2q "Voltage Rating [kV]"; p3_4q "Voltage initial guess [p.u.  rad]"; p5q "Area number"; p6q "Region number"
      mask help: Bus block.
      mask init:
      | fm_inout
      settings: AttributesFormatString="|V| =  1.05   p.u.\\n<V  = -0.4150 rad"
      mask CallbackString: ||||fm_block|
      mask Display: plot([0 1 1 0 0],[0 0 1 1 0])
  San Fernando II 230kV : PMComponent  Tag=PSATblock  Description=Connection  PhysicalDomain=psatdomain  LeftPortType=p1  RightPortType=p1  LConnTagsString=__newl0|__newl1  RConnTagsString=__newr0  mask(Bus){in=2, out=1, p2q=230, p3_4q=[1.0021    -0.55915], p5q=1, p6q=1}
      mask prompts: in "Number of inputs:"; out "Number of outputs:"; p2q "Voltage Rating [kV]"; p3_4q "Voltage initial guess [p.u.  rad]"; p5q "Area number"; p6q "Region number"
      mask help: Bus block.
      mask init:
      | fm_inout
      settings: AttributesFormatString="|V| =  1.0345 p.u.\\n<V  = -0.2868 rad"
      mask CallbackString: ||||fm_block|
      mask Display: plot([0 1 1 0 0],[0 0 1 1 0])
  San Geronimo 400kV : PMComponent  Tag=PSATblock  Description=Connection  PhysicalDomain=psatdomain  LeftPortType=p1  RightPortType=p1  LConnTagsString=__newl0|__newl1|__newl2|__newl3|__newl4  RConnTagsString=__newr0|__newr1|__newr2  mask(Bus){in=5, out=3, p2q=400, p3_4q=[1.0293    -0.26664], p5q=1, p6q=1}
      mask prompts: in "Number of inputs:"; out "Number of outputs:"; p2q "Voltage Rating [kV]"; p3_4q "Voltage initial guess [p.u.  rad]"; p5q "Area number"; p6q "Region number"
      mask help: Bus block.
      mask init:
      | fm_inout
      settings: AttributesFormatString="|V| =  1.0501 p.u.\\n<V  = -0.1354 rad"
      mask CallbackString: ||||fm_block|
      mask Display: plot([0 1 1 0 0],[0 0 1 1 0])
  San Geronimo 765kV : PMComponent  Tag=PSATblock  Description=Connection  PhysicalDomain=psatdomain  LeftPortType=p1  RightPortType=p1  LConnTagsString=__newl0|__newl1|__newl2|__newl3|__newl4  RConnTagsString=__newr0|__newr1|__newr2|__newr3|__newr4|__newr5  mask(Bus){in=5, out=6, p2q=765, p3_4q=[1.05     -0.2544], p5q=1, p6q=1}
      mask prompts: in "Number of inputs:"; out "Number of outputs:"; p2q "Voltage Rating [kV]"; p3_4q "Voltage initial guess [p.u.  rad]"; p5q "Area number"; p6q "Region number"
      mask help: Bus block.
      mask init:
      | fm_inout
      settings: AttributesFormatString="|V| =  1.05   p.u.\\n<V  = -0.1449 rad"
      mask CallbackString: ||||fm_block|
      mask Display: plot([0 1 1 0 0],[0 0 1 1 0])
  San Mateo (Colombia) : PMComponent  Tag=PSATblock  Description=Connection  PhysicalDomain=psatdomain  LeftPortType=p1  RightPortType=p1  LConnTagsString=__newl0  RConnTagsString=__newr0|__newr1  mask(Bus){in=1, out=2, p2q=230, p3_4q=[1.0593    -0.69162], p5q=1, p6q=1}
      mask prompts: in "Number of inputs:"; out "Number of outputs:"; p2q "Voltage Rating [kV]"; p3_4q "Voltage initial guess [p.u.  rad]"; p5q "Area number"; p6q "Region number"
      mask help: Bus block.
      mask init:
      | fm_inout
      settings: AttributesFormatString="|V| =  1.024  p.u.\\n<V  =  0.6391 rad"
      mask CallbackString: ||||fm_block|
      mask Display: plot([0 1 1 0 0],[0 0 1 1 0])
  Santa Elena : PMComponent  Tag=PSATblock  Description=Connection  PhysicalDomain=psatdomain  LeftPortType=p1  RightPortType=p1  LConnTagsString=__newl0|__newl1  RConnTagsString=__newr0  mask(Bus){in=2, out=1, p2q=230, p3_4q=[1.0158    -0.30624], p5q=1, p6q=1}
      mask prompts: in "Number of inputs:"; out "Number of outputs:"; p2q "Voltage Rating [kV]"; p3_4q "Voltage initial guess [p.u.  rad]"; p5q "Area number"; p6q "Region number"
      mask help: Bus block.
      mask init:
      | fm_inout
      settings: AttributesFormatString="|V| =  0.9926 p.u.\\n<V  = -0.3138 rad"
      mask CallbackString: ||||fm_block|
      mask Display: plot([0 1 1 0 0],[0 0 1 1 0])
  Santa Teresa 230kV : PMComponent  Tag=PSATblock  Description=Connection  PhysicalDomain=psatdomain  LeftPortType=p1  RightPortType=p1  LConnTagsString=__newl0|__newl1|__newl2|__newl3|__newl4|__newl5  RConnTagsString=__newr0|__newr1|__newr2|__newr3|__newr4  mask(Bus){in=6, out=5, p2q=230, p3_4q=[0.93698    -0.47554], p5q=1, p6q=1}
      mask prompts: in "Number of inputs:"; out "Number of outputs:"; p2q "Voltage Rating [kV]"; p3_4q "Voltage initial guess [p.u.  rad]"; p5q "Area number"; p6q "Region number"
      mask help: Bus block.
      mask init:
      | fm_inout
      settings: AttributesFormatString="|V| =  1.0049 p.u.\\n<V  = -0.2654 rad"
      mask CallbackString: ||||fm_block|
      mask Display: plot([0 1 1 0 0],[0 0 1 1 0])
  Santa Teresa 400kV : PMComponent  Tag=PSATblock  Description=Connection  PhysicalDomain=psatdomain  LeftPortType=p1  RightPortType=p1  LConnTagsString=__newl0|__newl1  RConnTagsString=__newr0|__newr1|__newr2|__newr3  mask(Bus){in=2, out=4, p2q=400, p3_4q=[0.90882     -0.3702], p5q=1, p6q=1}
      mask prompts: in "Number of inputs:"; out "Number of outputs:"; p2q "Voltage Rating [kV]"; p3_4q "Voltage initial guess [p.u.  rad]"; p5q "Area number"; p6q "Region number"
      mask help: Bus block.
      mask init:
      | fm_inout
      settings: AttributesFormatString="|V| =  1.033  p.u.\\n<V  = -0.2057 rad"
      mask CallbackString: ||||fm_block|
      mask Display: plot([0 1 1 0 0],[0 0 1 1 0])
  Shunt1 : PMComponent  Tag=PSATblock  Description=Power Flow  PhysicalDomain=psatdomain  LeftPortType=p1  RightPortType=p1  LConnTagsString=__newl0  mask(Shunt){p2_3_4q=[100  400  60], p6q=0.00125, p7q=on}
      mask prompts: p2_3_4q "Power, Voltage and Frequency Ratings [MVA, kV, Hz]"; p6q "Susceptance B [p.u.]"; p7q "Connected"
      mask help:
      | This block defines a static condenser:
      |
      | Q = B * V^2
      |
      | (Negative values of B define an inductive load).
      mask init:
      | fm_block
      mask CallbackString: ||fm_block
      mask Display: plot(-[0 60 60 55 53 55 60 60 55 53]/150,[0 0 8 16 25 16 8 -8 -16 -25]/50,-[80 80 80 150]/150,[25 -25 0 0]/50,[0 0],[-0.4 0.4],[0.075 0.075],[-0.25 0.25],[0.15 0.15],[-0.1 0.1])
  Shunt2 : PMComponent  Tag=PSATblock  Description=Power Flow  PhysicalDomain=psatdomain  LeftPortType=p1  RightPortType=p1  LConnTagsString=__newl0  mask(Shunt){p2_3_4q=[100  230  60], p6q=0.000675, p7q=on}
      mask prompts: p2_3_4q "Power, Voltage and Frequency Ratings [MVA, kV, Hz]"; p6q "Susceptance B [p.u.]"; p7q "Connected"
      mask help:
      | This block defines a static condenser:
      |
      | Q = B * V^2
      |
      | (Negative values of B define an inductive load).
      mask init:
      | fm_block
      mask CallbackString: ||fm_block
      mask Display: plot(-[0 60 60 55 53 55 60 60 55 53]/150,[0 0 8 16 25 16 8 -8 -16 -25]/50,-[80 80 80 150]/150,[25 -25 0 0]/50,[0 0],[-0.4 0.4],[0.075 0.075],[-0.25 0.25],[0.15 0.15],[-0.1 0.1])
  Shunt3 : PMComponent  Tag=PSATblock  Description=Power Flow  PhysicalDomain=psatdomain  LeftPortType=p1  RightPortType=p1  LConnTagsString=__newl0  mask(Shunt){p2_3_4q=[100  115  60], p6q=0.000907372, p7q=off}
      mask prompts: p2_3_4q "Power, Voltage and Frequency Ratings [MVA, kV, Hz]"; p6q "Susceptance B [p.u.]"; p7q "Connected"
      mask help:
      | This block defines a static condenser:
      |
      | Q = B * V^2
      |
      | (Negative values of B define an inductive load).
      mask init:
      | fm_block
      mask CallbackString: ||fm_block
      mask Display: plot(-[0 60 60 55 53 55 60 60 55 53]/150,[0 0 8 16 25 16 8 -8 -16 -25]/50,-[80 80 80 150]/150,[25 -25 0 0]/50,[0 0],[-0.4 0.4],[0.075 0.075],[-0.25 0.25],[0.15 0.15],[-0.1 0.1])
  Shunt4 : PMComponent  Tag=PSATblock  Description=Power Flow  PhysicalDomain=psatdomain  LeftPortType=p1  RightPortType=p1  LConnTagsString=__newl0  mask(Shunt){p2_3_4q=[100  230  60], p6q=[0.001512287], p7q=on}
      mask prompts: p2_3_4q "Power, Voltage and Frequency Ratings [MVA, kV, Hz]"; p6q "Susceptance B [p.u.]"; p7q "Connected"
      mask help:
      | This block defines a static condenser:
      |
      | Q = B * V^2
      |
      | (Negative values of B define an inductive load).
      mask init:
      | fm_block
      mask CallbackString: ||fm_block
      mask Display: plot(-[0 60 60 55 53 55 60 60 55 53]/150,[0 0 8 16 25 16 8 -8 -16 -25]/50,-[80 80 80 150]/150,[25 -25 0 0]/50,[0 0],[-0.4 0.4],[0.075 0.075],[-0.25 0.25],[0.15 0.15],[-0.1 0.1])
  Slack : PMComponent  Tag=PSATblock  Description=Power Flow  PhysicalDomain=psatdomain  LeftPortType=p1  RightPortType=p1  RConnTagsString=__newr0  mask(SW){p2_3q=[100  765], p4q=1.05, p5q=0.00, p6_7q=[1.5  -1.5], p8_9q=[1.1  0.9], p10q=30, p11q=1, p12q=on, p13q=on}
      mask prompts: p2_3q "Power and Voltage Ratings [MVA, kV]"; p4q "Voltage Magnitude [p.u.]"; p5q "Reference Phase Angle [rad]"; p6_7q "Qmax and Qmin [p.u.  p.u.]"; p8_9q "Vmax and Vmin  [p.u.  p.u.]"; p10q "Active Power Guess [p.u.]"; p11q "Loss Participation Factor"; p12q "Reference bus"; p13q "Connected"
      mask help:
      | This block defines a V-theta bus:
      |
      | V = V_des
      | theta = theta_des
      mask init:
      | [x,y] = fm_draw('circle');
      | [xt,yt] = fm_draw('theta');
      mask CallbackString: |||||||fm_block|fm_block
      mask Display: plot([0 1 1 0 0],[0 0 1 1 0]), color('blue'), plot([0 1],[0 1],[0 1],[1 0],[0.5 1 0.5 0 0.5],[0 0.5 1 0.5 0])
  Sur OMZ 230kV : PMComponent  Tag=PSATblock  Description=Connection  PhysicalDomain=psatdomain  LeftPortType=p1  RightPortType=p1  LConnTagsString=__newl0|__newl1|__newl2|__newl3  RConnTagsString=__newr0|__newr1  mask(Bus){in=4, out=2, p2q=230, p3_4q=[1.0224    -0.42388], p5q=1, p6q=1}
      mask prompts: in "Number of inputs:"; out "Number of outputs:"; p2q "Voltage Rating [kV]"; p3_4q "Voltage initial guess [p.u.  rad]"; p5q "Area number"; p6q "Region number"
      mask help: Bus block.
      mask init:
      | fm_inout
      settings: AttributesFormatString="|V| =  1.0352 p.u.\\n<V  = -0.2615 rad"
      mask CallbackString: ||||fm_block|
      mask Display: plot([0 1 1 0 0],[0 0 1 1 0])
  Sur OMZ 765kV : PMComponent  Tag=PSATblock  Description=Connection  PhysicalDomain=psatdomain  LeftPortType=p1  RightPortType=p1  LConnTagsString=__newl0|__newl1  RConnTagsString=__newr0|__newr1  mask(Bus){in=2, out=2, p2q=765, p3_4q=[1.0514    -0.36841], p5q=1, p6q=1}
      mask prompts: in "Number of inputs:"; out "Number of outputs:"; p2q "Voltage Rating [kV]"; p3_4q "Voltage initial guess [p.u.  rad]"; p5q "Area number"; p6q "Region number"
      mask help: Bus block.
      mask init:
      | fm_inout
      settings: AttributesFormatString="|V| =  1.0559 p.u.\\n<V  = -0.2191 rad"
      mask CallbackString: ||||fm_block|
      mask Display: plot([0 1 1 0 0],[0 0 1 1 0])
  Syn : Subsystem  Tag=PSATblock  Description=Machines  mask(Syn){p2_3_4q=[1044.4  138   60], p5q=6, p7_6q=[0.003125  0.15], p8_9_10q=[1.1 0.23 0.2], p11_12q=[6.5 0.035], p13_14_15q=[1.08 0.15 0.12], p16_17q=[1.25 0.035], p18_19q=[5 5], p20_21q=[20  0.00], p22_23q=[1.00  1.00], p24q=0.002, p25_26q=[1.07 1.18], in=1, p27q=1, p28q=on}
      mask prompts: p2_3_4q "Power, voltage and frequency ratings [MVA, kV, Hz]"; p5q "Machine Dynamic Order"; p7_6q "resistance ra and leakage reactance xl [p.u. p.u.]"; p8_9_10q "d-axis reactances Xd, X'd X"d [p.u.,p.u.,p.u.]"; p11_12q "d-axis open circuit time constants T'd0 and T"d0 [s, s]"; p13_14_15q "q-axis reactances Xq, X'q, X"q [p.u.  p.u.  p.u.]"; p16_17q "q-axis open circuit time constants T'q0 and T"q0 [s s]"; p18_19q "Inertia (M = 2H) and Damping [s, p.u.]"; p20_21q "Speed and active power additional signals Kw and Kp [p.u., p.u.]"; p22_23q "Percentage of active and reactive powers at bus [p.u. p.u.]"; p24q "d-axis additional circuit leakage time constant Taa [s]"; p25_26q "Saturation coefficients S(1.0) and S(1.2)"; in "Number of input signals"; p27q "COI number"; p28q "Connected"
      mask help: This block defines a fourth order synchronous machine.
      mask init:
      | fm_inout
      | [x,y] = fm_draw('circle');
      | [xg,yg] = fm_draw('G');
      | [xs,ys] = fm_draw('sinus');
      mask StyleString: edit,popup(8|6|5.3|5.2|5.1|4|3|2),edit,edit,edit,edit,edit,edit,edit,edit,edit,edit,popup(0|1|2),edit,checkbox
      mask CallbackString: |fm_block|||||||||||||fm_block
      mask Display:
      | plot(x+1.4,y,0.12*xs+1,0.15*ys-0.6)
      | color('blue')
      | plot(1.4+0.45*xg,0.3+0.45*yg)
  Syn1 : Subsystem  Tag=PSATblock  Description=Machines  mask(Syn){p2_3_4q=[700  765   60], p5q=6, p7_6q=[0.00591975  0.11], p8_9_10q=[0.92 0.315 0.255], p11_12q=[9.1 0.03], p13_14_15q=[0.62 0.62 0.33], p16_17q=[3.7 0.05], p18_19q=[2.4 5], p20_21q=[0.00  0.00], p22_23q=[1.00  1.00], p24q=0.002, p25_26q=[1.07 1.18], in=2, p27q=1, p28q=on}
      mask prompts: p2_3_4q "Power, voltage and frequency ratings [MVA, kV, Hz]"; p5q "Machine Dynamic Order"; p7_6q "resistance ra and leakage reactance xl [p.u. p.u.]"; p8_9_10q "d-axis reactances Xd, X'd X"d [p.u.,p.u.,p.u.]"; p11_12q "d-axis open circuit time constants T'd0 and T"d0 [s, s]"; p13_14_15q "q-axis reactances Xq, X'q, X"q [p.u.  p.u.  p.u.]"; p16_17q "q-axis open circuit time constants T'q0 and T"q0 [s s]"; p18_19q "Inertia (M = 2H) and Damping [s, p.u.]"; p20_21q "Speed and active power additional signals Kw and Kp [p.u., p.u.]"; p22_23q "Percentage of active and reactive powers at bus [p.u. p.u.]"; p24q "d-axis additional circuit leakage time constant Taa [s]"; p25_26q "Saturation coefficients S(1.0) and S(1.2)"; in "Number of input signals"; p27q "COI number"; p28q "Connected"
      mask help: This block defines a fourth order synchronous machine.
      mask init:
      | fm_inout
      | [x,y] = fm_draw('circle');
      | [xg,yg] = fm_draw('G');
      | [xs,ys] = fm_draw('sinus');
      mask StyleString: edit,popup(8|6|5.3|5.2|5.1|4|3|2),edit,edit,edit,edit,edit,edit,edit,edit,edit,edit,popup(0|1|2),edit,checkbox
      mask CallbackString: |fm_block|||||||||||||fm_block
      mask Display:
      | plot(x+1.4,y,0.12*xs+1,0.15*ys-0.6)
      | color('blue')
      | plot(1.4+0.45*xg,0.3+0.45*yg)
  Syn10 : Subsystem  Tag=PSATblock  Description=Machines  mask(Syn){p2_3_4q=[204  115   60], p5q=6, p7_6q=[0.003125  0.15], p8_9_10q=[1.48 0.16 0.12], p11_12q=[10 0.035], p13_14_15q=[1.48 0.16 0.12], p16_17q=[1.25 0.035], p18_19q=[5 5], p20_21q=[25  0.00], p22_23q=[1.00  1.00], p24q=0.002, p25_26q=[1.07 1.18], in=1, p27q=1, p28q=on}
      mask prompts: p2_3_4q "Power, voltage and frequency ratings [MVA, kV, Hz]"; p5q "Machine Dynamic Order"; p7_6q "resistance ra and leakage reactance xl [p.u. p.u.]"; p8_9_10q "d-axis reactances Xd, X'd X"d [p.u.,p.u.,p.u.]"; p11_12q "d-axis open circuit time constants T'd0 and T"d0 [s, s]"; p13_14_15q "q-axis reactances Xq, X'q, X"q [p.u.  p.u.  p.u.]"; p16_17q "q-axis open circuit time constants T'q0 and T"q0 [s s]"; p18_19q "Inertia (M = 2H) and Damping [s, p.u.]"; p20_21q "Speed and active power additional signals Kw and Kp [p.u., p.u.]"; p22_23q "Percentage of active and reactive powers at bus [p.u. p.u.]"; p24q "d-axis additional circuit leakage time constant Taa [s]"; p25_26q "Saturation coefficients S(1.0) and S(1.2)"; in "Number of input signals"; p27q "COI number"; p28q "Connected"
      mask help: This block defines a fourth order synchronous machine.
      mask init:
      | fm_inout
      | [x,y] = fm_draw('circle');
      | [xg,yg] = fm_draw('G');
      | [xs,ys] = fm_draw('sinus');
      mask StyleString: edit,popup(8|6|5.3|5.2|5.1|4|3|2),edit,edit,edit,edit,edit,edit,edit,edit,edit,edit,popup(0|1|2),edit,checkbox
      mask CallbackString: |fm_block|||||||||||||fm_block
      mask Display:
      | plot(x+1.4,y,0.12*xs+1,0.15*ys-0.6)
      | color('blue')
      | plot(1.4+0.45*xg,0.3+0.45*yg)
  Syn11 : Subsystem  Tag=PSATblock  Description=Machines  mask(Syn){p2_3_4q=[333  230   60], p5q=6, p7_6q=[0.003125  0.15], p8_9_10q=[1.48 0.16 0.12], p11_12q=[10 0.035], p13_14_15q=[1.48 0.16 0.12], p16_17q=[1.25 0.035], p18_19q=[5 5], p20_21q=[25  0.00], p22_23q=[1.00  1.00], p24q=0.002, p25_26q=[1.07 1.18], in=1, p27q=1, p28q=on}
      mask prompts: p2_3_4q "Power, voltage and frequency ratings [MVA, kV, Hz]"; p5q "Machine Dynamic Order"; p7_6q "resistance ra and leakage reactance xl [p.u. p.u.]"; p8_9_10q "d-axis reactances Xd, X'd X"d [p.u.,p.u.,p.u.]"; p11_12q "d-axis open circuit time constants T'd0 and T"d0 [s, s]"; p13_14_15q "q-axis reactances Xq, X'q, X"q [p.u.  p.u.  p.u.]"; p16_17q "q-axis open circuit time constants T'q0 and T"q0 [s s]"; p18_19q "Inertia (M = 2H) and Damping [s, p.u.]"; p20_21q "Speed and active power additional signals Kw and Kp [p.u., p.u.]"; p22_23q "Percentage of active and reactive powers at bus [p.u. p.u.]"; p24q "d-axis additional circuit leakage time constant Taa [s]"; p25_26q "Saturation coefficients S(1.0) and S(1.2)"; in "Number of input signals"; p27q "COI number"; p28q "Connected"
      mask help: This block defines a fourth order synchronous machine.
      mask init:
      | fm_inout
      | [x,y] = fm_draw('circle');
      | [xg,yg] = fm_draw('G');
      | [xs,ys] = fm_draw('sinus');
      mask StyleString: edit,popup(8|6|5.3|5.2|5.1|4|3|2),edit,edit,edit,edit,edit,edit,edit,edit,edit,edit,popup(0|1|2),edit,checkbox
      mask CallbackString: |fm_block|||||||||||||fm_block
      mask Display:
      | plot(x+1.4,y,0.12*xs+1,0.15*ys-0.6)
      | color('blue')
      | plot(1.4+0.45*xg,0.3+0.45*yg)
  Syn2 : Subsystem  Tag=PSATblock  Description=Machines  mask(Syn){p2_3_4q=[733  138   60], p5q=6, p7_6q=[0.003125  0.15], p8_9_10q=[1.1 0.23 0.2], p11_12q=[1.024 0.025], p13_14_15q=[1.08 0.15 0.12], p16_17q=[1.0024 0.025], p18_19q=[5 5], p20_21q=[25  0.00], p22_23q=[1.00  1.00], p24q=0.002, p25_26q=[1.07 1.18], in=1, p27q=1, p28q=on}
      mask prompts: p2_3_4q "Power, voltage and frequency ratings [MVA, kV, Hz]"; p5q "Machine Dynamic Order"; p7_6q "resistance ra and leakage reactance xl [p.u. p.u.]"; p8_9_10q "d-axis reactances Xd, X'd X"d [p.u.,p.u.,p.u.]"; p11_12q "d-axis open circuit time constants T'd0 and T"d0 [s, s]"; p13_14_15q "q-axis reactances Xq, X'q, X"q [p.u.  p.u.  p.u.]"; p16_17q "q-axis open circuit time constants T'q0 and T"q0 [s s]"; p18_19q "Inertia (M = 2H) and Damping [s, p.u.]"; p20_21q "Speed and active power additional signals Kw and Kp [p.u., p.u.]"; p22_23q "Percentage of active and reactive powers at bus [p.u. p.u.]"; p24q "d-axis additional circuit leakage time constant Taa [s]"; p25_26q "Saturation coefficients S(1.0) and S(1.2)"; in "Number of input signals"; p27q "COI number"; p28q "Connected"
      mask help: This block defines a fourth order synchronous machine.
      mask init:
      | fm_inout
      | [x,y] = fm_draw('circle');
      | [xg,yg] = fm_draw('G');
      | [xs,ys] = fm_draw('sinus');
      mask StyleString: edit,popup(8|6|5.3|5.2|5.1|4|3|2),edit,edit,edit,edit,edit,edit,edit,edit,edit,edit,popup(0|1|2),edit,checkbox
      mask CallbackString: |fm_block|||||||||||||fm_block
      mask Display:
      | plot(x+1.4,y,0.12*xs+1,0.15*ys-0.6)
      | color('blue')
      | plot(1.4+0.45*xg,0.3+0.45*yg)
  Syn3 : Subsystem  Tag=PSATblock  Description=Machines  mask(Syn){p2_3_4q=[440  400   60], p5q=6, p7_6q=[0.003125  0.15], p8_9_10q=[1.1 0.23 0.2], p11_12q=[1.024 0.025], p13_14_15q=[1.08 0.15 0.12], p16_17q=[1.0024 0.025], p18_19q=[5 5], p20_21q=[20  0.00], p22_23q=[1.00  1.00], p24q=0.002, p25_26q=[1.07 1.18], in=1, p27q=1, p28q=on}
      mask prompts: p2_3_4q "Power, voltage and frequency ratings [MVA, kV, Hz]"; p5q "Machine Dynamic Order"; p7_6q "resistance ra and leakage reactance xl [p.u. p.u.]"; p8_9_10q "d-axis reactances Xd, X'd X"d [p.u.,p.u.,p.u.]"; p11_12q "d-axis open circuit time constants T'd0 and T"d0 [s, s]"; p13_14_15q "q-axis reactances Xq, X'q, X"q [p.u.  p.u.  p.u.]"; p16_17q "q-axis open circuit time constants T'q0 and T"q0 [s s]"; p18_19q "Inertia (M = 2H) and Damping [s, p.u.]"; p20_21q "Speed and active power additional signals Kw and Kp [p.u., p.u.]"; p22_23q "Percentage of active and reactive powers at bus [p.u. p.u.]"; p24q "d-axis additional circuit leakage time constant Taa [s]"; p25_26q "Saturation coefficients S(1.0) and S(1.2)"; in "Number of input signals"; p27q "COI number"; p28q "Connected"
      mask help: This block defines a fourth order synchronous machine.
      mask init:
      | fm_inout
      | [x,y] = fm_draw('circle');
      | [xg,yg] = fm_draw('G');
      | [xs,ys] = fm_draw('sinus');
      mask StyleString: edit,popup(8|6|5.3|5.2|5.1|4|3|2),edit,edit,edit,edit,edit,edit,edit,edit,edit,edit,popup(0|1|2),edit,checkbox
      mask CallbackString: |fm_block|||||||||||||fm_block
      mask Display:
      | plot(x+1.4,y,0.12*xs+1,0.15*ys-0.6)
      | color('blue')
      | plot(1.4+0.45*xg,0.3+0.45*yg)
  Syn4 : Subsystem  Tag=PSATblock  Description=Machines  mask(Syn){p2_3_4q=[220  400   60], p5q=6, p7_6q=[0.00229167  0.11], p8_9_10q=[0.8 0.184 0.14], p11_12q=[5.6 0.03], p13_14_15q=[0.48 0.14 0.14], p16_17q=[3.7 0.05], p18_19q=[2.4 5], p20_21q=[20  0.00], p22_23q=[1.00  1.00], p24q=0.002, p25_26q=[1.07 1.18], in=1, p27q=1, p28q=on}
      mask prompts: p2_3_4q "Power, voltage and frequency ratings [MVA, kV, Hz]"; p5q "Machine Dynamic Order"; p7_6q "resistance ra and leakage reactance xl [p.u. p.u.]"; p8_9_10q "d-axis reactances Xd, X'd X"d [p.u.,p.u.,p.u.]"; p11_12q "d-axis open circuit time constants T'd0 and T"d0 [s, s]"; p13_14_15q "q-axis reactances Xq, X'q, X"q [p.u.  p.u.  p.u.]"; p16_17q "q-axis open circuit time constants T'q0 and T"q0 [s s]"; p18_19q "Inertia (M = 2H) and Damping [s, p.u.]"; p20_21q "Speed and active power additional signals Kw and Kp [p.u., p.u.]"; p22_23q "Percentage of active and reactive powers at bus [p.u. p.u.]"; p24q "d-axis additional circuit leakage time constant Taa [s]"; p25_26q "Saturation coefficients S(1.0) and S(1.2)"; in "Number of input signals"; p27q "COI number"; p28q "Connected"
      mask help: This block defines a fourth order synchronous machine.
      mask init:
      | fm_inout
      | [x,y] = fm_draw('circle');
      | [xg,yg] = fm_draw('G');
      | [xs,ys] = fm_draw('sinus');
      mask StyleString: edit,popup(8|6|5.3|5.2|5.1|4|3|2),edit,edit,edit,edit,edit,edit,edit,edit,edit,edit,popup(0|1|2),edit,checkbox
      mask CallbackString: |fm_block|||||||||||||fm_block
      mask Display:
      | plot(x+1.4,y,0.12*xs+1,0.15*ys-0.6)
      | color('blue')
      | plot(1.4+0.45*xg,0.3+0.45*yg)
  Syn5 : Subsystem  Tag=PSATblock  Description=Machines  mask(Syn){p2_3_4q=[240  400   60], p5q=6, p7_6q=[0.00229167  0.11], p8_9_10q=[0.8 0.184 0.14], p11_12q=[5.6 0.03], p13_14_15q=[0.48 0.14 0.14], p16_17q=[3.7 0.05], p18_19q=[2.4 5], p20_21q=[20  0.00], p22_23q=[1.00  1.00], p24q=0.002, p25_26q=[1.07 1.18], in=1, p27q=1, p28q=on}
      mask prompts: p2_3_4q "Power, voltage and frequency ratings [MVA, kV, Hz]"; p5q "Machine Dynamic Order"; p7_6q "resistance ra and leakage reactance xl [p.u. p.u.]"; p8_9_10q "d-axis reactances Xd, X'd X"d [p.u.,p.u.,p.u.]"; p11_12q "d-axis open circuit time constants T'd0 and T"d0 [s, s]"; p13_14_15q "q-axis reactances Xq, X'q, X"q [p.u.  p.u.  p.u.]"; p16_17q "q-axis open circuit time constants T'q0 and T"q0 [s s]"; p18_19q "Inertia (M = 2H) and Damping [s, p.u.]"; p20_21q "Speed and active power additional signals Kw and Kp [p.u., p.u.]"; p22_23q "Percentage of active and reactive powers at bus [p.u. p.u.]"; p24q "d-axis additional circuit leakage time constant Taa [s]"; p25_26q "Saturation coefficients S(1.0) and S(1.2)"; in "Number of input signals"; p27q "COI number"; p28q "Connected"
      mask help: This block defines a fourth order synchronous machine.
      mask init:
      | fm_inout
      | [x,y] = fm_draw('circle');
      | [xg,yg] = fm_draw('G');
      | [xs,ys] = fm_draw('sinus');
      mask StyleString: edit,popup(8|6|5.3|5.2|5.1|4|3|2),edit,edit,edit,edit,edit,edit,edit,edit,edit,edit,popup(0|1|2),edit,checkbox
      mask CallbackString: |fm_block|||||||||||||fm_block
      mask Display:
      | plot(x+1.4,y,0.12*xs+1,0.15*ys-0.6)
      | color('blue')
      | plot(1.4+0.45*xg,0.3+0.45*yg)
  Syn6 : Subsystem  Tag=PSATblock  Description=Machines  mask(Syn){p2_3_4q=[333.3  230   60], p5q=6, p7_6q=[0.00229167  0.11], p8_9_10q=[0.82 0.28 0.21], p11_12q=[5.6 0.03], p13_14_15q=[0.45 0.21 0.21], p16_17q=[3.7 0.05], p18_19q=[2.4 5], p20_21q=[20  0.00], p22_23q=[1.00  1.00], p24q=0.002, p25_26q=[1.07 1.18], in=1, p27q=1, p28q=on}
      mask prompts: p2_3_4q "Power, voltage and frequency ratings [MVA, kV, Hz]"; p5q "Machine Dynamic Order"; p7_6q "resistance ra and leakage reactance xl [p.u. p.u.]"; p8_9_10q "d-axis reactances Xd, X'd X"d [p.u.,p.u.,p.u.]"; p11_12q "d-axis open circuit time constants T'd0 and T"d0 [s, s]"; p13_14_15q "q-axis reactances Xq, X'q, X"q [p.u.  p.u.  p.u.]"; p16_17q "q-axis open circuit time constants T'q0 and T"q0 [s s]"; p18_19q "Inertia (M = 2H) and Damping [s, p.u.]"; p20_21q "Speed and active power additional signals Kw and Kp [p.u., p.u.]"; p22_23q "Percentage of active and reactive powers at bus [p.u. p.u.]"; p24q "d-axis additional circuit leakage time constant Taa [s]"; p25_26q "Saturation coefficients S(1.0) and S(1.2)"; in "Number of input signals"; p27q "COI number"; p28q "Connected"
      mask help: This block defines a fourth order synchronous machine.
      mask init:
      | fm_inout
      | [x,y] = fm_draw('circle');
      | [xg,yg] = fm_draw('G');
      | [xs,ys] = fm_draw('sinus');
      mask StyleString: edit,popup(8|6|5.3|5.2|5.1|4|3|2),edit,edit,edit,edit,edit,edit,edit,edit,edit,edit,popup(0|1|2),edit,checkbox
      mask CallbackString: |fm_block|||||||||||||fm_block
      mask Display:
      | plot(x+1.4,y,0.12*xs+1,0.15*ys-0.6)
      | color('blue')
      | plot(1.4+0.45*xg,0.3+0.45*yg)
  Syn7 : Subsystem  Tag=PSATblock  Description=Machines  mask(Syn){p2_3_4q=[266.7  230   60], p5q=6, p7_6q=[0.00229167  0.11], p8_9_10q=[0.82 0.28 0.21], p11_12q=[5.6 0.03], p13_14_15q=[0.45 0.21 0.21], p16_17q=[3.7 0.05], p18_19q=[2.4 5], p20_21q=[20  0.00], p22_23q=[1.00  1.00], p24q=0.002, p25_26q=[1.07 1.18], in=1, p27q=1, p28q=on}
      mask prompts: p2_3_4q "Power, voltage and frequency ratings [MVA, kV, Hz]"; p5q "Machine Dynamic Order"; p7_6q "resistance ra and leakage reactance xl [p.u. p.u.]"; p8_9_10q "d-axis reactances Xd, X'd X"d [p.u.,p.u.,p.u.]"; p11_12q "d-axis open circuit time constants T'd0 and T"d0 [s, s]"; p13_14_15q "q-axis reactances Xq, X'q, X"q [p.u.  p.u.  p.u.]"; p16_17q "q-axis open circuit time constants T'q0 and T"q0 [s s]"; p18_19q "Inertia (M = 2H) and Damping [s, p.u.]"; p20_21q "Speed and active power additional signals Kw and Kp [p.u., p.u.]"; p22_23q "Percentage of active and reactive powers at bus [p.u. p.u.]"; p24q "d-axis additional circuit leakage time constant Taa [s]"; p25_26q "Saturation coefficients S(1.0) and S(1.2)"; in "Number of input signals"; p27q "COI number"; p28q "Connected"
      mask help: This block defines a fourth order synchronous machine.
      mask init:
      | fm_inout
      | [x,y] = fm_draw('circle');
      | [xg,yg] = fm_draw('G');
      | [xs,ys] = fm_draw('sinus');
      mask StyleString: edit,popup(8|6|5.3|5.2|5.1|4|3|2),edit,edit,edit,edit,edit,edit,edit,edit,edit,edit,popup(0|1|2),edit,checkbox
      mask CallbackString: |fm_block|||||||||||||fm_block
      mask Display:
      | plot(x+1.4,y,0.12*xs+1,0.15*ys-0.6)
      | color('blue')
      | plot(1.4+0.45*xg,0.3+0.45*yg)
  Syn8 : Subsystem  Tag=PSATblock  Description=Machines  mask(Syn){p2_3_4q=[503  230   60], p5q=6, p7_6q=[0.003125  0.15], p8_9_10q=[1.939 0.277 0.2522], p11_12q=[1.024 0.025], p13_14_15q=[1.939 0.277 0.2143], p16_17q=[1.024 0.025], p18_19q=[5 5], p20_21q=[20  0.00], p22_23q=[1.00  1.00], p24q=0.002, p25_26q=[1.07 1.18], in=1, p27q=1, p28q=on}
      mask prompts: p2_3_4q "Power, voltage and frequency ratings [MVA, kV, Hz]"; p5q "Machine Dynamic Order"; p7_6q "resistance ra and leakage reactance xl [p.u. p.u.]"; p8_9_10q "d-axis reactances Xd, X'd X"d [p.u.,p.u.,p.u.]"; p11_12q "d-axis open circuit time constants T'd0 and T"d0 [s, s]"; p13_14_15q "q-axis reactances Xq, X'q, X"q [p.u.  p.u.  p.u.]"; p16_17q "q-axis open circuit time constants T'q0 and T"q0 [s s]"; p18_19q "Inertia (M = 2H) and Damping [s, p.u.]"; p20_21q "Speed and active power additional signals Kw and Kp [p.u., p.u.]"; p22_23q "Percentage of active and reactive powers at bus [p.u. p.u.]"; p24q "d-axis additional circuit leakage time constant Taa [s]"; p25_26q "Saturation coefficients S(1.0) and S(1.2)"; in "Number of input signals"; p27q "COI number"; p28q "Connected"
      mask help: This block defines a fourth order synchronous machine.
      mask init:
      | fm_inout
      | [x,y] = fm_draw('circle');
      | [xg,yg] = fm_draw('G');
      | [xs,ys] = fm_draw('sinus');
      mask StyleString: edit,popup(8|6|5.3|5.2|5.1|4|3|2),edit,edit,edit,edit,edit,edit,edit,edit,edit,edit,popup(0|1|2),edit,checkbox
      mask CallbackString: |fm_block|||||||||||||fm_block
      mask Display:
      | plot(x+1.4,y,0.12*xs+1,0.15*ys-0.6)
      | color('blue')
      | plot(1.4+0.45*xg,0.3+0.45*yg)
  Syn9 : Subsystem  Tag=PSATblock  Description=Machines  mask(Syn){p2_3_4q=[203.5  115   60], p5q=6, p7_6q=[0.003125  0.15], p8_9_10q=[1.65 0.275 0.185], p11_12q=[6.5 0.035], p13_14_15q=[1.65 0.5 0.185], p16_17q=[1.25 0.035], p18_19q=[5 5], p20_21q=[25  0.00], p22_23q=[1.00  1.00], p24q=0.002, p25_26q=[1.07 1.18], in=1, p27q=1, p28q=on}
      mask prompts: p2_3_4q "Power, voltage and frequency ratings [MVA, kV, Hz]"; p5q "Machine Dynamic Order"; p7_6q "resistance ra and leakage reactance xl [p.u. p.u.]"; p8_9_10q "d-axis reactances Xd, X'd X"d [p.u.,p.u.,p.u.]"; p11_12q "d-axis open circuit time constants T'd0 and T"d0 [s, s]"; p13_14_15q "q-axis reactances Xq, X'q, X"q [p.u.  p.u.  p.u.]"; p16_17q "q-axis open circuit time constants T'q0 and T"q0 [s s]"; p18_19q "Inertia (M = 2H) and Damping [s, p.u.]"; p20_21q "Speed and active power additional signals Kw and Kp [p.u., p.u.]"; p22_23q "Percentage of active and reactive powers at bus [p.u. p.u.]"; p24q "d-axis additional circuit leakage time constant Taa [s]"; p25_26q "Saturation coefficients S(1.0) and S(1.2)"; in "Number of input signals"; p27q "COI number"; p28q "Connected"
      mask help: This block defines a fourth order synchronous machine.
      mask init:
      | fm_inout
      | [x,y] = fm_draw('circle');
      | [xg,yg] = fm_draw('G');
      | [xs,ys] = fm_draw('sinus');
      mask StyleString: edit,popup(8|6|5.3|5.2|5.1|4|3|2),edit,edit,edit,edit,edit,edit,edit,edit,edit,edit,popup(0|1|2),edit,checkbox
      mask CallbackString: |fm_block|||||||||||||fm_block
      mask Display:
      | plot(x+1.4,y,0.12*xs+1,0.15*ys-0.6)
      | color('blue')
      | plot(1.4+0.45*xg,0.3+0.45*yg)
  Tacoa 230kV : PMComponent  Tag=PSATblock  Description=Connection  PhysicalDomain=psatdomain  LeftPortType=p1  RightPortType=p1  LConnTagsString=__newl0|__newl1|__newl2|__newl3  RConnTagsString=__newr0|__newr1  mask(Bus){in=4, out=2, p2q=230, p3_4q=[1.05    -0.45942], p5q=1, p6q=1}
      mask prompts: in "Number of inputs:"; out "Number of outputs:"; p2q "Voltage Rating [kV]"; p3_4q "Voltage initial guess [p.u.  rad]"; p5q "Area number"; p6q "Region number"
      mask help: Bus block.
      mask init:
      | fm_inout
      settings: AttributesFormatString="|V| =  1.05   p.u.\\n<V  = -0.2850 rad"
      mask CallbackString: ||||fm_block|
      mask Display: plot([0 1 1 0 0],[0 0 1 1 0])
  Termobarrancas : PMComponent  Tag=PSATblock  Description=Connection  PhysicalDomain=psatdomain  LeftPortType=p1  RightPortType=p1  LConnTagsString=__newl0  RConnTagsString=__newr0  mask(Bus){in=1, out=1, p2q=230, p3_4q=[1.0585     -0.6092], p5q=1, p6q=1}
      mask prompts: in "Number of inputs:"; out "Number of outputs:"; p2q "Voltage Rating [kV]"; p3_4q "Voltage initial guess [p.u.  rad]"; p5q "Area number"; p6q "Region number"
      mask help: Bus block.
      mask init:
      | fm_inout
      settings: AttributesFormatString="|V| =  1.05   p.u.\\n<V  = -0.2132 rad"
      mask CallbackString: ||||fm_block|
      mask Display: plot([0 1 1 0 0],[0 0 1 1 0])
  Tg2 : Subsystem  Tag=PSATblock  Description=Controls  mask(Tg){p2q=2, p3q=1.00, p4q=0.00001, p5q=10, p6q=0, p7q=6, p8q=36, p9q=0.00, p10q=12.00, p11q=50.00, p12q=on}
      mask prompts: p2q "Turbine governor type"; p3q "Reference speed [p.u.]"; p4q "Droop R [p.u./p.u.]"; p5q "Maximum torque [p.u.]"; p6q "Minimum torque [p.u.]"; p7q "Pole Time Constant T2 [s]"; p8q "Zero Time Constant T1 [s]"; p9q "Transient gain time constant T3 [s]"; p10q "Power fraction time constant T4 [s]"; p11q "Reheat time constant T5 [s]"; p12q "Connected"
      mask help: This block defines a Turbine Governor.
      mask init:
      | [x,y] = fm_draw('G');
      mask Help:
      | This block defines  a Turbine Governor.
      | There are two kind of regulators:
      | 
      | Type 1:
      | 
      |      IEEE Model 4
      | 
      | Type 2:
      | 
      |      IEEE Model 1
      mask StyleString: popup(1|2),edit,edit,edit,edit,edit,edit,edit,edit,edit,checkbox
      mask CallbackString: fm_block||||||||||fm_block
      mask Display:
      | plot([-1.8 2.8 2.8 -1.8 -1.8],[-1.5 -1.5 1.5 1.5 -1.5])
      | color('red')
      | plot([-0.5 -0.5],[-1 1],[-1.3 0.3],[1 1])
      | plot(1.4+x,y)
  Tiara 230kV : PMComponent  Tag=PSATblock  Description=Connection  PhysicalDomain=psatdomain  LeftPortType=p1  RightPortType=p1  LConnTagsString=__newl0|__newl1  RConnTagsString=__newr0  mask(Bus){in=2, out=1, p2q=230, p3_4q=[0.95955    -0.48769], p5q=1, p6q=1}
      mask prompts: in "Number of inputs:"; out "Number of outputs:"; p2q "Voltage Rating [kV]"; p3_4q "Voltage initial guess [p.u.  rad]"; p5q "Area number"; p6q "Region number"
      mask help: Bus block.
      mask init:
      | fm_inout
      settings: AttributesFormatString="|V| =  1.0077 p.u.\\n<V  = -0.2882 rad"
      mask CallbackString: ||||fm_block|
      mask Display: plot([0 1 1 0 0],[0 0 1 1 0])
  Trinidad 138kV : PMComponent  Tag=PSATblock  Description=Connection  PhysicalDomain=psatdomain  LeftPortType=p1  RightPortType=p1  LConnTagsString=__newl0|__newl1|__newl2  RConnTagsString=__newr0|__newr1  mask(Bus){in=3, out=2, p2q=138, p3_4q=[1.0329    -0.91001], p5q=1, p6q=1}
      mask prompts: in "Number of inputs:"; out "Number of outputs:"; p2q "Voltage Rating [kV]"; p3_4q "Voltage initial guess [p.u.  rad]"; p5q "Area number"; p6q "Region number"
      mask help: Bus block.
      mask init:
      | fm_inout
      settings: AttributesFormatString="|V| =  1.02   p.u.\\n<V  = -0.3452 rad"
      mask CallbackString: ||||fm_block|
      mask Display: plot([0 1 1 0 0],[0 0 1 1 0])
  Trinidad 230kV : PMComponent  Tag=PSATblock  Description=Connection  PhysicalDomain=psatdomain  LeftPortType=p1  RightPortType=p1  LConnTagsString=__newl0  RConnTagsString=__newr0  mask(Bus){in=1, out=1, p2q=230, p3_4q=[0.99849    -0.84504], p5q=1, p6q=1}
      mask prompts: in "Number of inputs:"; out "Number of outputs:"; p2q "Voltage Rating [kV]"; p3_4q "Voltage initial guess [p.u.  rad]"; p5q "Area number"; p6q "Region number"
      mask help: Bus block.
      mask init:
      | fm_inout
      settings: AttributesFormatString="|V| =  1.0321 p.u.\\n<V  = -0.3658 rad"
      mask CallbackString: ||||fm_block|
      mask Display: plot([0 1 1 0 0],[0 0 1 1 0])
  Urdaneta 138kV : PMComponent  Tag=PSATblock  Description=Connection  PhysicalDomain=psatdomain  LeftPortType=p1  RightPortType=p1  LConnTagsString=__newl0|__newl1|__newl2  RConnTagsString=__newr0|__newr1  mask(Bus){in=3, out=2, p2q=138, p3_4q=[1.07    -0.87735], p5q=1, p6q=1}
      mask prompts: in "Number of inputs:"; out "Number of outputs:"; p2q "Voltage Rating [kV]"; p3_4q "Voltage initial guess [p.u.  rad]"; p5q "Area number"; p6q "Region number"
      mask help: Bus block.
      mask init:
      | fm_inout
      settings: AttributesFormatString="|V| =  1.05   p.u.\\n<V  = -0.2267 rad"
      mask CallbackString: ||||fm_block|
      mask Display: plot([0 1 1 0 0],[0 0 1 1 0])
  Uribante 230kV : PMComponent  Tag=PSATblock  Description=Connection  PhysicalDomain=psatdomain  LeftPortType=p1  RightPortType=p1  LConnTagsString=__newl0|__newl1|__newl2|__newl3  RConnTagsString=__newr0|__newr1|__newr2  mask(Bus){in=4, out=3, p2q=230, p3_4q=[1.0674    -0.65301], p5q=1, p6q=1}
      mask prompts: in "Number of inputs:"; out "Number of outputs:"; p2q "Voltage Rating [kV]"; p3_4q "Voltage initial guess [p.u.  rad]"; p5q "Area number"; p6q "Region number"
      mask help: Bus block.
      mask init:
      | fm_inout
      settings: AttributesFormatString="|V| =  1.0365 p.u.\\n<V  =  0.6829 rad"
      mask CallbackString: ||||fm_block|
      mask Display: plot([0 1 1 0 0],[0 0 1 1 0])
  Valencia 230kV : PMComponent  Tag=PSATblock  Description=Connection  PhysicalDomain=psatdomain  LeftPortType=p1  RightPortType=p1  LConnTagsString=__newl0  RConnTagsString=__newr0|__newr1|__newr2  mask(Bus){in=1, out=3, p2q=230, p3_4q=[0.94798    -0.58922], p5q=1, p6q=1}
      mask prompts: in "Number of inputs:"; out "Number of outputs:"; p2q "Voltage Rating [kV]"; p3_4q "Voltage initial guess [p.u.  rad]"; p5q "Area number"; p6q "Region number"
      mask help: Bus block.
      mask init:
      | fm_inout
      settings: AttributesFormatString="|V| =  0.9684 p.u.\\n<V  = -0.3702 rad"
      mask CallbackString: ||||fm_block|
      mask Display: plot([0 1 1 0 0],[0 0 1 1 0])
  Varname : fm_lib/Connections/Varname  Tag=PSATblock  Description=OPF & CPF  SystemSampleTime=-1  pxq="[1  2  7  8  13  14  19  20  25  26  31  32  37  38  43  44  49  50  55  56  61  62  67  68  76  80  84  88  92  96  100  104  108  112  116  120  189  293  300  304  332  338  349  352  356  360  364  368  372  376  380  523]"
  Yaracuy 230kV : PMComponent  Tag=PSATblock  Description=Connection  PhysicalDomain=psatdomain  LeftPortType=p1  RightPortType=p1  LConnTagsString=__newl0|__newl1|__newl2|__newl3  RConnTagsString=__newr0|__newr1|__newr2|__newr3|__newr4|__newr5  mask(Bus){in=4, out=6, p2q=230, p3_4q=[0.9567      -0.546], p5q=1, p6q=1}
      mask prompts: in "Number of inputs:"; out "Number of outputs:"; p2q "Voltage Rating [kV]"; p3_4q "Voltage initial guess [p.u.  rad]"; p5q "Area number"; p6q "Region number"
      mask help: Bus block.
      mask init:
      | fm_inout
      settings: AttributesFormatString="|V| =  0.9894 p.u.\\n<V  = -0.3171 rad"
      mask CallbackString: ||||fm_block|
      mask Display: plot([0 1 1 0 0],[0 0 1 1 0])
  Yaracuy 400kV : PMComponent  Tag=PSATblock  Description=Connection  PhysicalDomain=psatdomain  LeftPortType=p1  RightPortType=p1  LConnTagsString=__newl0|__newl1|__newl2|__newl3  RConnTagsString=__newr0|__newr1|__newr2|__newr3  mask(Bus){in=4, out=4, p2q=400, p3_4q=[0.94273    -0.52379], p5q=1, p6q=1}
      mask prompts: in "Number of inputs:"; out "Number of outputs:"; p2q "Voltage Rating [kV]"; p3_4q "Voltage initial guess [p.u.  rad]"; p5q "Area number"; p6q "Region number"
      mask help: Bus block.
      mask init:
      | fm_inout
      settings: AttributesFormatString="|V| =  1.0008 p.u.\\n<V  = -0.2802 rad"
      mask CallbackString: ||||fm_block|
      mask Display: plot([0 1 1 0 0],[0 0 1 1 0])
  Yaracuy 765kV : PMComponent  Tag=PSATblock  Description=Connection  PhysicalDomain=psatdomain  LeftPortType=p1  RightPortType=p1  LConnTagsString=__newl0|__newl1|__newl2  RConnTagsString=__newr0|__newr1|__newr2|__newr3  mask(Bus){in=3, out=4, p2q=765, p3_4q=[0.98704    -0.46859], p5q=1, p6q=1}
      mask prompts: in "Number of inputs:"; out "Number of outputs:"; p2q "Voltage Rating [kV]"; p3_4q "Voltage initial guess [p.u.  rad]"; p5q "Area number"; p6q "Region number"
      mask help: Bus block.
      mask init:
      | fm_inout
      settings: AttributesFormatString="|V| =  1.0128 p.u.\\n<V  = -0.2712 rad"
      mask CallbackString: ||||fm_block|
      mask Display: plot([0 1 1 0 0],[0 0 1 1 0])
  wires:
  AVR1/1(Out1) -> Syn1/1(in_1)
  Tg2/1(Out1) -> Syn1/2(in_2)
  AVR5/1(Out1) -> Syn4/1(in_1)
  AVR6/1(Out1) -> Syn5/1(in_1)
  AVR4/1(Out1) -> Syn8/1(in_1)
  AVR12/1(Out1) -> Syn11/1(in_1)
  AVR10/1(Out1) -> Syn9/1(in_1)
  AVR3/1(Out1) -> Syn/1(in_1)
  Pss/1(Out1) -> AVR3/1(in_1)
  AVR2/1(Out1) -> Syn2/1(in_1)
  AVR13/1(Out1) -> Syn3/1(in_1)
  AVR8/1(Out1) -> Syn6/1(in_1)
  AVR7/1(Out1) -> Syn7/1(in_1)
  Pss1/1(Out1) -> AVR8/1(in_1)
  AVR11/1(Out1) -> Syn10/1(in_1)
  connections:
  Guri 765kV/LConn6 -- Auto/LConn1
  Guri 765kV/LConn5 -- Auto1/LConn1
  Guri 765kV/LConn4 -- Auto2/LConn1
  Auto3/RConn1 -- Guri 230kV/LConn1
  El Tigre 400kV/LConn1 -- Line22/LConn1
  El Tigre 400kV/LConn2 -- Line27/LConn1
  La Canoa 400kV/LConn1 -- Line17/LConn1
  La Canoa 400kV/LConn2 -- Line16/RConn1
  Auto4/RConn1 -- San Geronimo 400kV/LConn1
  Auto5/RConn1 -- San Geronimo 400kV/LConn2
  El Tigre 400kV/LConn3 -- Auto7/LConn1
  El Tigre 400kV/LConn4 -- Auto6/LConn1
  Line6/RConn1 -- Macagua II/LConn3
  Guayana B/LConn1 -- Line9/LConn1
  Guayana B/LConn2 -- Line47/LConn1
  Line9/RConn1 -- Macagua II/LConn1
  Line47/RConn1 -- Macagua II/LConn2
  Line105/LConn1 -- Guri 230kV/LConn3
  Line19/LConn1 -- Guri 230kV/LConn2
  Line152/RConn1 -- Ciudad Bolivar 230kV/RConn1
  Line36/RConn1 -- Ciudad Bolivar 230kV/LConn1
  Malena/LConn1 -- Line3/RConn1
  Malena/LConn2 -- Line4/RConn1
  Malena/LConn3 -- Line5/RConn1
  San Geronimo 765kV/LConn5 -- Auto4/LConn1
  San Geronimo 765kV/LConn4 -- Auto5/LConn1
  Guri 400kV B/LConn1 -- Auto/RConn1
  Guri 400kV B/LConn2 -- Auto1/RConn1
  Guri 400kV B/LConn3 -- Auto2/RConn1
  Guri 400kV A/LConn6 -- Auto3/LConn1
  Guri 400kV A/LConn5 -- Line7/LConn1
  Guri 400kV A/LConn4 -- Line101/LConn1
  Guri 400kV A/LConn3 -- Line18/LConn1
  Guri 400kV A/LConn2 -- Line16/LConn1
  Guri 400kV B/LConn4 -- Auto61/LConn1
  Auto61/RConn1 -- Guri 400kV A/LConn1
  Line144/LConn1 -- Guri 400kV B/RConn3
  Line157/RConn1 -- Guri 400kV B/RConn1
  Line15/RConn1 -- Guri 400kV B/RConn2
  Guayana B/RConn1 -- Line15/LConn1
  Guayana B/RConn2 -- Line157/LConn1
  Line8/LConn1 -- Guayana B/LConn3
  Line19/RConn1 -- Guayana A/RConn1
  Line105/RConn1 -- Guayana A/RConn2
  Guayana A/LConn1 -- Line152/LConn1
  El Tigre 230kV/LConn6 -- Line36/LConn1
  El Tigre 230kV/LConn5 -- Line25/LConn1
  Line56/LConn1 -- Guayana A/LConn2
  Line56/RConn1 -- Ciudad Bolivar 230kV/RConn2
  Ciudad Bolivar 230kV/LConn2 -- Line25/RConn1
  Auto6/RConn1 -- El Tigre 230kV/RConn3
  Auto7/RConn1 -- El Tigre 230kV/RConn2
  PQ46/LConn1 -- Malena/RConn1
  PQ68/LConn1 -- El Tigre 230kV/RConn4
  Slack/RConn1 -- Guri 765kV/RConn1
  PQ32/LConn1 -- Ciudad Bolivar 230kV/RConn3
  PQ29/LConn1 -- Guayana A/LConn4
  Line27/RConn1 -- San Geronimo 400kV/RConn3
  Line22/RConn1 -- San Geronimo 400kV/RConn2
  PQ28/LConn1 -- San Geronimo 400kV/RConn1
  PQ34/LConn1 -- El Tigre 230kV/RConn1
  Guayana B/LConn4 -- PQ36/LConn1
  PV12/RConn1 -- Guayana A/LConn3
  PV9/RConn1 -- Guri 400kV A/RConn1
  Caruachi/LConn2 -- PV11/RConn1
  PV8/RConn1 -- Guri 230kV/RConn1
  Syn1/RConn1 -- Guri 765kV/RConn2
  Syn4/RConn1 -- Caruachi/LConn3
  Macagua II/RConn2 -- PV14/RConn1
  Syn5/RConn1 -- Macagua II/RConn3
  PQ43/LConn1 -- San Geronimo 765kV/RConn6
  SC1/RConn1 -- San Geronimo 765kV/RConn5
  Line5/LConn1 -- San Geronimo 765kV/RConn4
  Line4/LConn1 -- San Geronimo 765kV/RConn3
  Line3/LConn1 -- San Geronimo 765kV/RConn2
  Guri 765kV/LConn1 -- Line/RConn1
  Guri 765kV/LConn2 -- Line1/RConn1
  Guri 765kV/LConn3 -- Line2/RConn1
  Line101/RConn1 -- El Tigre 400kV/RConn4
  Line18/RConn1 -- El Tigre 400kV/RConn3
  Line17/RConn1 -- El Tigre 400kV/RConn2
  Line183/RConn1 -- El Tigre 400kV/RConn1
  Line183/LConn1 -- Gen. Anz 2012-2/RConn1
  Line13/LConn1 -- Furrial 400kV/LConn1
  Line7/RConn1 -- Palital 400kV/RConn2
  Palital 400kV/LConn1 -- Line13/RConn1
  Line8/RConn1 -- Palital 400kV/RConn1
  Palital 400kV/LConn2 -- Line73/RConn1
  Line73/LConn1 -- Furrial 400kV/LConn2
  Auto73/LConn1 -- Furrial 400kV/RConn1
  Auto73/RConn1 -- Furrial 230kV/RConn3
  Furrial 230kV/RConn2 -- Line99/LConn1
  Furrial 230kV/RConn1 -- Line30/LConn1
  Furrial 400kV/RConn2 -- PQ12/LConn1
  Palital 400kV/LConn3 -- PQ31/LConn1
  El Tigre 230kV/LConn1 -- Line31/LConn1
  El Tigre 230kV/LConn2 -- Line28/LConn1
  Line146/LConn1 -- El Tigre 400kV/LConn5
  Jose 400kV/LConn2 -- Line23/RConn1
  San Geronimo 400kV/LConn3 -- Line23/LConn1
  Shunt1/LConn1 -- Jose 400kV/RConn3
  El Tigre 230kV/LConn3 -- Line74/LConn1
  El Tigre 230kV/LConn4 -- Line34/LConn1
  Line34/RConn1 -- Furrial 230kV/LConn2
  Line74/RConn1 -- Furrial 230kV/LConn1
  Line146/RConn1 -- Barbacoa II 400kV/LConn2
  Barbacoa II 400kV/RConn1 -- Auto11/LConn1
  Jose 400kV/LConn1 -- Line147/LConn1
  Line147/RConn1 -- Barbacoa II 400kV/LConn1
  Barbacoa II 230kV/RConn1 -- Auto11/RConn1
  Santa Teresa 400kV/RConn1 -- Line35/RConn1
  Line20/RConn1 -- Santa Teresa 400kV/RConn2
  Line20/LConn1 -- San Geronimo 400kV/LConn5
  Ciudad Losada 400kV/LConn1 -- Line38/LConn1
  Line38/RConn1 -- Santa Teresa 400kV/RConn3
  Auto20/RConn1 -- Santa Teresa 230kV/LConn2
  Auto19/RConn1 -- Santa Teresa 230kV/LConn1
  Sur OMZ 765kV/LConn1 -- Auto22/LConn1
  Sur OMZ 765kV/LConn2 -- Auto21/LConn1
  Auto22/RConn1 -- Sur OMZ 230kV/RConn1
  Auto21/RConn1 -- Sur OMZ 230kV/RConn2
  Santa Teresa 400kV/LConn1 -- Auto20/LConn1
  Santa Teresa 400kV/LConn2 -- Auto19/LConn1
  Line39/LConn1 -- Sur OMZ 765kV/RConn2
  Line40/LConn1 -- Sur OMZ 765kV/RConn1
  Sur OMZ 230kV/LConn4 -- Line14/LConn1
  Sur OMZ 230kV/LConn3 -- Line26/LConn1
  Line26/RConn1 -- Papelon 230kV/RConn1
  Line14/RConn1 -- Papelon 230kV/RConn2
  Line46/RConn1 -- Junquito 230kV/RConn1
  Line10/RConn1 -- Junquito 230kV/RConn2
  Line10/LConn1 -- Sur OMZ 230kV/LConn2
  Sur OMZ 230kV/LConn1 -- Line46/LConn1
  Santa Teresa 230kV/LConn3 -- Line164/LConn1
  Line164/RConn1 -- Papelon 230kV/RConn3
  Santa Teresa 230kV/LConn4 -- Line50/LConn1
  Line48/RConn1 -- Papelon 230kV/LConn1
  Line45/RConn1 -- Boyaca 230kV/LConn1
  Line54/RConn1 -- Convento 230kV/LConn1
  Line53/RConn1 -- Convento 230kV/LConn2
  Junquito 230kV/LConn3 -- Line48/LConn1
  Boyaca 230kV/LConn2 -- Line54/LConn1
  Line50/RConn1 -- Convento 230kV/LConn3
  Auto24/RConn1 -- La Horqueta 230kV/LConn1
  Auto17/RConn1 -- Ciudad Losada 230kV/LConn1
  Ciudad Losada 230kV/RConn2 -- Line66/LConn1
  Ciudad Losada 230kV/RConn1 -- Line63/LConn1
  Line67/RConn1 -- La Horqueta 230kV/RConn4
  Line158/RConn1 -- Santa Teresa 230kV/RConn1
  Line21/RConn1 -- Santa Teresa 230kV/RConn2
  Line33/RConn1 -- Santa Teresa 230kV/RConn4
  Line32/RConn1 -- Santa Teresa 230kV/RConn3
  Barbacoa II 230kV/LConn2 -- Line24/LConn1
  Barbacoa II 230kV/LConn1 -- Line72/LConn1
  Rio Chico II/LConn1 -- Line37/LConn1
  Rio Chico II/RConn1 -- Line33/LConn1
  Line28/RConn1 -- Barbacoa I 230kV/LConn3
  Line31/RConn1 -- Barbacoa I 230kV/LConn2
  Barbacoa II 230kV/LConn3 -- Line55/LConn1
  Line29/LConn1 -- Barbacoa II 230kV/LConn4
  Line66/RConn1 -- La Horqueta 230kV/RConn5
  Auto26/RConn1 -- La Horqueta 230kV/RConn1
  Auto25/RConn1 -- La Horqueta 230kV/LConn2
  La Horqueta 230kV/LConn5 -- Line76/LConn1
  La Horqueta 230kV/LConn6 -- Line80/LConn1
  La Horqueta 230kV/LConn7 -- Line78/LConn1
  La Horqueta 230kV/LConn8 -- Line98/LConn1
  Line98/RConn1 -- Macaro 230kV/RConn2
  Line78/RConn1 -- Macaro 230kV/RConn1
  Line82/RConn1 -- Macaro 230kV/LConn1
  Macaro 230kV/LConn2 -- Line81/RConn1
  San Geronimo 765kV/LConn3 -- Line39/RConn1
  Ciudad Losada 230kV/LConn3 -- Line158/LConn1
  Ciudad Losada 230kV/LConn2 -- Line21/LConn1
  PQ61/LConn1 -- Santa Teresa 400kV/RConn4
  Santa Teresa 230kV/RConn5 -- Line71/LConn1
  Line71/RConn1 -- Barbacoa I 230kV/RConn1
  Line37/RConn1 -- Barbacoa I 230kV/RConn2
  Line72/RConn1 -- Barbacoa I 230kV/RConn3
  Line24/RConn1 -- Barbacoa I 230kV/RConn4
  Junquito 230kV/LConn1 -- Line52/LConn1
  Line52/RConn1 -- Tacoa 230kV/RConn1
  Macaro 230kV/LConn3 -- PQ22/LConn1
  Junquito 230kV/LConn2 -- PQ39/LConn1
  PQ41/LConn1 -- Tacoa 230kV/RConn2
  PQ42/LConn1 -- Boyaca 230kV/RConn1
  PQ44/LConn1 -- Convento 230kV/RConn1
  Papelon 230kV/LConn2 -- PQ40/LConn1
  Rio Chico II/LConn2 -- PQ14/LConn1
  Ciudad Losada 230kV/LConn4 -- PQ26/LConn1
  Tacoa 230kV/LConn1 -- PV2/RConn1
  Santa Teresa 230kV/LConn5 -- PQ27/LConn1
  San Geronimo 400kV/LConn4 -- Line35/LConn1
  PQ33/LConn1 -- Jose 400kV/RConn1
  Barbacoa I 230kV/LConn1 -- PQ13/LConn1
  Tacoa 230kV/LConn4 -- Line45/LConn1
  Tacoa 230kV/LConn3 -- Line53/LConn1
  Tacoa 230kV/LConn2 -- Syn8/RConn1
  Santa Teresa 230kV/LConn6 -- Line179/LConn1
  Line179/RConn1 -- Gen. Miranda 2012/RConn1
  Jose 400kV/RConn2 -- Line182/RConn1
  Gen. Anz 2012-1/RConn1 -- Line182/LConn1
  La Horqueta 765kV/RConn3 -- Line40/RConn1
  Line140/LConn1 -- La Horqueta 765kV/RConn1
  Line44/LConn1 -- La Horqueta 765kV/RConn2
  Auto23/LConn1 -- La Horqueta 765kV/LConn1
  Auto26/LConn1 -- La Horqueta 765kV/LConn2
  Line140/RConn1 -- La Arenosa 765kV/RConn4
  Ciudad Losada 400kV/RConn1 -- Auto17/LConn1
  Tiara 230kV/LConn2 -- Line63/RConn1
  Tiara 230kV/LConn1 -- Line67/LConn1
  La Arenosa 765kV/LConn1 -- Auto28/LConn1
  La Arenosa 765kV/LConn2 -- Auto27/LConn1
  Auto23/RConn1 -- La Horqueta 400kV/RConn2
  Line77/RConn1 -- La Horqueta 230kV/LConn3
  Line89/RConn1 -- La Horqueta 230kV/LConn4
  Aragua 230kV/LConn2 -- Line76/RConn1
  Aragua 230kV/LConn1 -- Line80/RConn1
  Line79/RConn1 -- Aragua 230kV/RConn2
  Caña de Azucar 230kV/LConn2 -- Line82/LConn1
  Caña de Azucar 230kV/LConn1 -- Line83/RConn1
  La Horqueta 400kV/LConn4 -- Auto24/LConn1
  La Horqueta 400kV/LConn3 -- Auto25/LConn1
  Line64/RConn1 -- La Horqueta 400kV/LConn2
  Line70/RConn1 -- La Horqueta 400kV/LConn1
  San Diego 230kV/LConn4 -- Line83/LConn1
  San Diego 230kV/LConn3 -- Line81/LConn1
  La Arenosa 400kV/LConn6 -- Auto29/LConn1
  La Arenosa 400kV/LConn5 -- Line64/LConn1
  La Arenosa 400kV/LConn4 -- Line70/LConn1
  Line87/RConn1 -- San Diego 230kV/LConn1
  Line94/RConn1 -- San Diego 230kV/LConn2
  Auto29/RConn1 -- La Arenosa 230kV/LConn1
  San Geronimo 765kV/LConn2 -- Line44/RConn1
  La Arenosa 230kV/RConn5 -- Line110/RConn1
  La Arenosa 230kV/RConn7 -- Line94/LConn1
  La Arenosa 230kV/RConn6 -- Line87/LConn1
  Auto28/RConn1 -- La Arenosa 230kV/RConn1
  Auto27/RConn1 -- La Arenosa 230kV/RConn2
  La Arenosa 230kV/LConn8 -- Line79/LConn1
  La Arenosa 230kV/LConn7 -- Line65/LConn1
  La Arenosa 230kV/LConn6 -- Line77/LConn1
  La Arenosa 230kV/LConn5 -- Line89/LConn1
  Line88/LConn1 -- La Arenosa 230kV/LConn4
  Line86/LConn1 -- La Arenosa 230kV/LConn3
  PQ4/LConn1 -- La Arenosa 765kV/RConn5
  La Horqueta 400kV/RConn1 -- PQ65/LConn1
  La Arenosa 400kV/RConn1 -- PQ66/LConn1
  La Horqueta 765kV/RConn4 -- SC3/RConn1
  Aragua 230kV/RConn3 -- Line32/LConn1
  PQ21/LConn1 -- Caña de Azucar 230kV/RConn1
  PQ18/LConn1 -- La Arenosa 230kV/RConn8
  PQ19/LConn1 -- San Diego 230kV/RConn1
  Aragua 230kV/LConn3 -- PQ20/LConn1
  Line108/RConn1 -- La Horqueta 230kV/RConn3
  Line107/RConn1 -- La Horqueta 230kV/RConn2
  San Fernando II 230kV/LConn1 -- Line109/LConn1
  PQ25/LConn1 -- San Fernando II 230kV/RConn1
  PV13/RConn1 -- San Diego 230kV/RConn2
  Line65/RConn1 -- Aragua 230kV/RConn1
  PQ17/LConn1 -- Valencia 230kV/LConn1
  Syn11/RConn1 -- San Diego 230kV/RConn3
  San Geronimo 765kV/LConn1 -- Line43/RConn1
  Line43/LConn1 -- La Arenosa 765kV/RConn3
  Line109/RConn1 -- Calabozo 230kV/RConn1
  Calabozo 230kV/LConn3 -- Line108/LConn1
  Calabozo 230kV/LConn2 -- Line107/LConn1
  Line88/RConn1 -- Valencia 230kV/RConn3
  Line86/RConn1 -- Valencia 230kV/RConn2
  PQ24/LConn1 -- Calabozo 230kV/RConn3
  Line174/LConn1 -- San Fernando II 230kV/LConn2
  Line174/RConn1 -- Calabozo 230kV/RConn2
  Line178/RConn1 -- Calabozo 230kV/LConn1
  Line178/LConn1 -- Gen. Guarico 2012/RConn1
  PV6/RConn1 -- Guanta II 230kV/RConn1
  Guanta II 230kV/LConn1 -- Auto9/LConn1
  Auto9/RConn1 -- Guanta II 115kV/RConn1
  Guanta II 115kV/LConn1 -- Line154/RConn1
  Guanta II 115kV/LConn2 -- Line162/RConn1
  Guanta II 230kV/LConn2 -- PQ69/LConn1
  Line29/RConn1 -- Guanta II 230kV/RConn4
  Line55/RConn1 -- Guanta II 230kV/RConn3
  Cumana III/LConn2 -- Line165/LConn1
  Cumana III/LConn1 -- Line166/RConn1
  PQ71/LConn1 -- Cumana III/RConn1
  El Indio 230kV/LConn2 -- Line100/LConn1
  El Indio 230kV/LConn1 -- Line155/LConn1
  Line30/RConn1 -- El Indio 230kV/RConn1
  Line99/RConn1 -- El Indio 230kV/RConn2
  Line155/RConn1 -- Casanay 230kV/RConn3
  Line100/RConn1 -- Casanay 230kV/RConn4
  Casanay 230kV/RConn2 -- Line75/RConn1
  Casanay 230kV/RConn1 -- Line151/RConn1
  PQ59/LConn1 -- El Indio 230kV/RConn3
  PQ35/LConn1 -- El Indio 230kV/LConn3
  Line162/LConn1 -- Cumana II/LConn3
  Line154/LConn1 -- Cumana II/LConn2
  Guanta II 230kV/LConn4 -- Line75/LConn1
  Guanta II 230kV/LConn3 -- Line151/LConn1
  Line165/RConn1 -- Cumana II/LConn1
  Line166/LConn1 -- Manzanares/LConn1
  Cumana II/RConn1 -- Line167/RConn1
  Line167/LConn1 -- Manzanares/LConn2
  Casanay 230kV/LConn1 -- Auto8/LConn1
  Auto8/RConn1 -- Casanay 115kV/LConn1
  Cariaco/LConn1 -- Line168/RConn1
  Cumana II/RConn2 -- Line169/RConn1
  Line169/LConn1 -- Cariaco/RConn1
  Line168/LConn1 -- Casanay 115kV/RConn2
  Cumana II/RConn3 -- Line170/RConn1
  Line170/LConn1 -- Casanay 115kV/RConn1
  PQ57/LConn1 -- Cumana II/RConn4
  Manzanares/RConn1 -- PQ70/LConn1
  Cariaco/LConn2 -- PQ72/LConn1
  PQ47/LConn1 -- Casanay 115kV/LConn2
  Gen. Miranda 2012/LConn1 -- PV15/RConn1
  PV16/RConn1 -- Gen. Anz 2012-2/LConn1
  PV17/RConn1 -- Gen. Anz 2012-1/LConn1
  Gen. Guarico 2012/LConn1 -- PV18/RConn1
  Casanay 115kV/RConn3 -- Line171/RConn1
  Casanay 115kV/RConn4 -- Line172/RConn1
  Chicopata/LConn1 -- Line171/LConn1
  Line172/LConn1 -- Chicopata/LConn2
  Chicopata/RConn1 -- Line156/RConn1
  Luisa Caceres/LConn3 -- PQ73/LConn1
  Luisa Caceres/LConn2 -- PV/RConn1
  Luisa Caceres/LConn1 -- Syn9/RConn1
  Line156/LConn1 -- Luisa Caceres/RConn2
  Line11/RConn1 -- El Callao II 400kV/RConn1
  Macagua II/RConn1 -- Line11/LConn1
  Auto66/RConn1 -- Las Claritas 230kV/RConn1
  Auto66/LConn1 -- Las Claritas 400kV/LConn2
  Las Claritas 400kV/RConn1 -- Line12/RConn1
  Line12/LConn1 -- El Callao II 400kV/RConn2
  Las Claritas 230kV/LConn1 -- Line148/LConn1
  PQ67/LConn1 -- Las Claritas 400kV/LConn1
  El Callao II 400kV/LConn1 -- PQ30/LConn1
  Line148/RConn1 -- Santa Elena/RConn1
  Santa Elena/LConn1 -- Line149/LConn1
  Line149/RConn1 -- Boa Vista (Brasil)/RConn1
  PQ60/LConn1 -- Santa Elena/LConn2
  PQ1/LConn1 -- Boa Vista (Brasil)/LConn1
  PV10/RConn1 -- Urdaneta 138kV/RConn1
  Syn/RConn1 -- Urdaneta 138kV/RConn2
  PV5/RConn1 -- Ramon Laguna 138kV/RConn1
  Ramon Laguna 138kV/RConn2 -- Syn2/RConn1
  La Arenosa 400kV/RConn2 -- Line95/RConn1
  Line41/LConn1 -- La Arenosa 765kV/RConn1
  Auto37/RConn1 -- Planta Centro 230kV/LConn1
  La Arenosa 230kV/RConn3 -- Line92/LConn1
  La Arenosa 230kV/RConn4 -- Line163/LConn1
  Yaracuy 765kV/LConn1 -- Auto38/LConn1
  Yaracuy 765kV/LConn2 -- Auto39/LConn1
  Auto38/RConn1 -- Yaracuy 400kV/RConn4
  Auto39/RConn1 -- Yaracuy 230kV/RConn1
  Yaracuy 400kV/LConn4 -- Auto40/LConn1
  Auto40/RConn1 -- Yaracuy 230kV/LConn1
  Line95/LConn1 -- Yaracuy 400kV/RConn3
  Yaracuy 400kV/RConn2 -- Line91/LConn1
  La Arenosa 400kV/LConn2 -- Line85/LConn1
  La Arenosa 400kV/LConn1 -- Line90/LConn1
  Line106/RConn1 -- Cabudare 230kV/RConn2
  Line96/RConn1 -- Cabudare 230kV/RConn3
  Line84/RConn1 -- Yaracuy 230kV/RConn6
  Line122/RConn1 -- Yaracuy 230kV/RConn5
  Auto72/RConn1 -- Yaracuy 230kV/RConn2
  Yaracuy 765kV/LConn3 -- Auto72/LConn1
  La Arenosa 230kV/LConn2 -- Line93/LConn1
  PQ62/LConn1 -- Yaracuy 400kV/RConn1
  Cabudare 230kV/LConn1 -- Line110/LConn1
  PQ45/LConn1 -- Planta Centro 230kV/RConn6
  Yaracuy 230kV/LConn2 -- Line106/LConn1
  Yaracuy 230kV/LConn3 -- Line96/LConn1
  Yaracuy 230kV/LConn4 -- PQ49/LConn1
  PQ16/LConn1 -- Cabudare 230kV/RConn1
  Line93/RConn1 -- Planta Centro 230kV/RConn5
  Line92/RConn1 -- Planta Centro 230kV/RConn4
  Line163/RConn1 -- Planta Centro 230kV/RConn3
  PQ2/LConn1 -- Yaracuy 765kV/RConn2
  Yaracuy 765kV/RConn4 -- Line41/RConn1
  Yaracuy 765kV/RConn3 -- Line42/RConn1
  Planta Centro 400kV/LConn2 -- Syn3/RConn1
  Planta Centro 400kV/LConn1 -- PV7/RConn1
  Line42/LConn1 -- La Arenosa 765kV/RConn2
  PQ54/LConn1 -- P. Piedra 138kV/LConn1
  Line127/RConn1 -- P. Iguana/RConn1
  P. Iguana/LConn1 -- Line133/RConn1
  PQ37/LConn1 -- Cuatricentenario 138kV/LConn1
  P. Piedra 230kV/RConn1 -- Line133/LConn1
  Auto58/RConn1 -- P. Piedra 138kV/RConn1
  P. Piedra 230kV/LConn1 -- Auto58/LConn1
  El Rincon 138kV/LConn2 -- PQ53/LConn1
  PQ55/LConn1 -- Urdaneta 138kV/LConn3
  Line135/RConn1 -- Urdaneta 138kV/LConn1
  Line136/RConn1 -- Urdaneta 138kV/LConn2
  El Rincon 138kV/LConn1 -- Line139/RConn1
  Auto59/RConn1 -- El Rincon 138kV/RConn1
  Line104/RConn1 -- Morochas 230kV/RConn4
  Line103/RConn1 -- Morochas 230kV/RConn3
  Line102/RConn1 -- Morochas 230kV/RConn2
  Line103/LConn1 -- Yaracuy 230kV/RConn4
  Yaracuy 230kV/RConn3 -- Line104/LConn1
  PQ58/LConn1 -- Morochas 230kV/RConn1
  Shunt2/LConn1 -- Morochas 230kV/RConn5
  Morochas 230kV/LConn3 -- PQ7/LConn1
  Yaracuy 400kV/LConn3 -- Line60/LConn1
  Line59/LConn1 -- Yaracuy 400kV/LConn2
  Line97/LConn1 -- Yaracuy 400kV/LConn1
  Morochas 230kV/LConn1 -- Line113/LConn1
  Morochas 230kV/LConn2 -- Line114/LConn1
  Auto49/RConn1 -- El Tablazo 230kV/LConn1
  Line113/RConn1 -- El Tablazo 230kV/RConn1
  El Tablazo 400kV/LConn3 -- Auto49/LConn1
  El Tablazo 400kV/LConn1 -- Line123/LConn1
  El Tablazo 400kV/LConn2 -- Line49/LConn1
  El Tablazo 230kV/LConn2 -- Line126/LConn1
  El Tablazo 230kV/LConn3 -- Line58/LConn1
  Line126/RConn1 -- P. Palmas/RConn1
  Line58/RConn1 -- P. Palmas/RConn2
  P. Palmas/LConn1 -- Line129/RConn1
  P. Palmas/LConn2 -- Line57/RConn1
  Line114/RConn1 -- Cabimas 230kV/RConn2
  Cabimas 230kV/RConn1 -- Line112/LConn1
  El Tablazo 230kV/RConn2 -- Line112/RConn1
  PQ63/LConn1 -- El Tablazo 400kV/RConn1
  El Tablazo 230kV/LConn4 -- Line127/LConn1
  PQ5/LConn1 -- El Tablazo 230kV/LConn5
  Line97/RConn1 -- El Tablazo 400kV/RConn2
  Line59/RConn1 -- El Tablazo 400kV/RConn3
  Line60/RConn1 -- El Tablazo 400kV/RConn4
  Cabimas 230kV/LConn2 -- PQ8/LConn1
  Auto56/RConn1 -- Cuatricentenario 230kV/LConn1
  Line123/RConn1 -- Cuatricentenario 400kV/RConn1
  Line49/RConn1 -- Cuatricentenario 400kV/RConn2
  Peonias/LConn1 -- Line125/LConn1
  Cuatricentenario 230kV/RConn1 -- Line125/RConn1
  Cuatricentenario 230kV/RConn2 -- Line51/RConn1
  Line51/LConn1 -- Peonias/LConn2
  Line129/LConn1 -- Peonias/RConn1
  Line57/LConn1 -- Peonias/RConn2
  Cuatricentenario 400kV/LConn1 -- Auto56/LConn1
  Cuestecita (Colombia)/LConn1 -- Line138/LConn1
  Auto60/RConn1 -- Cuatricentenario 138kV/RConn1
  Cuatricentenario 230kV/LConn5 -- Auto60/LConn1
  Cuatricentenario 230kV/LConn4 -- Line134/LConn1
  Cuatricentenario 230kV/LConn3 -- Line131/LConn1
  Line138/RConn1 -- Cuatricentenario 230kV/LConn2
  El Rincon 138kV/RConn3 -- Line128/LConn1
  Line128/RConn1 -- Ramon Laguna 138kV/LConn4
  Trinidad 138kV/RConn2 -- Line137/LConn1
  Auto57/RConn1 -- Trinidad 138kV/RConn1
  Trinidad 138kV/LConn3 -- Line139/LConn1
  Trinidad 230kV/LConn1 -- Auto57/LConn1
  El Rincon 230kV/LConn1 -- Auto59/LConn1
  Line137/RConn1 -- Ramon Laguna 138kV/LConn2
  PQ52/LConn1 -- Trinidad 138kV/LConn1
  Line130/RConn1 -- Ramon Laguna 138kV/LConn5
  P. Piedra 138kV/RConn2 -- Line130/LConn1
  Line132/RConn1 -- Trinidad 138kV/LConn2
  Line131/RConn1 -- Trinidad 230kV/RConn1
  Line124/LConn1 -- El Rincon 138kV/RConn2
  Line134/RConn1 -- El Rincon 230kV/RConn1
  Line124/RConn1 -- Ramon Laguna 138kV/LConn3
  Cuatricentenario 138kV/RConn2 -- Line132/LConn1
  PQ51/LConn1 -- Ramon Laguna 138kV/LConn1
  Termobarrancas/LConn1 -- Line161/LConn1
  Line161/RConn1 -- Barinas IV 230kV/RConn1
  Las Flores 230kV/LConn1 -- Line143/LConn1
  Line68/RConn1 -- Barinas IV 230kV/LConn1
  Barinas IV 230kV/LConn2 -- Line141/RConn1
  Barinas IV 230kV/LConn3 -- Line120/LConn1
  Line120/RConn1 -- Las Flores 230kV/RConn1
  PQ11/LConn1 -- Barinas IV 230kV/LConn5
  Las Flores 230kV/LConn2 -- PQ3/LConn1
  Uribante 230kV/LConn1 -- Line117/RConn1
  Line118/RConn1 -- Planta Paez 230kV/RConn1
  Uribante 230kV/LConn2 -- Line116/LConn1
  Line116/RConn1 -- San Agaton/RConn1
  Uribante 230kV/LConn3 -- Line61/LConn1
  Line61/RConn1 -- San Agaton/RConn2
  Line160/RConn1 -- Uribante 230kV/RConn1
  Line69/RConn1 -- Uribante 230kV/RConn2
  Line141/LConn1 -- Planta Paez 230kV/RConn3
  Line68/LConn1 -- Planta Paez 230kV/RConn2
  PV3/RConn1 -- Planta Paez 230kV/LConn1
  PQ10/LConn1 -- Uribante 230kV/LConn4
  PV4/RConn1 -- San Agaton/LConn1
  Shunt4/LConn1 -- El Corozo 230kV/RConn4
  PQ9/LConn1 -- El Corozo 230kV/RConn1
  El Corozo 230kV/LConn1 -- Line160/LConn1
  El Corozo 230kV/LConn2 -- Line69/LConn1
  Line115/RConn1 -- El Corozo 230kV/RConn3
  Line111/RConn1 -- El Corozo 230kV/RConn2
  San Agaton/LConn2 -- Syn6/RConn1
  Planta Paez 230kV/LConn3 -- PQ23/LConn1
  Planta Paez 230kV/LConn2 -- Syn7/RConn1
  Buena Vista 230kV/LConn1 -- Line102/LConn1
  Line62/RConn1 -- Buena Vista 230kV/RConn1
  El Vigia II 230kV/LConn1 -- Line62/LConn1
  Line118/LConn1 -- Buena Vista 230kV/RConn2
  Buena Vista 230kV/LConn2 -- PQ38/LConn1
  El Vigia II 230kV/LConn2 -- PQ6/LConn1
  San Mateo (Colombia)/RConn1 -- Line111/LConn1
  San Mateo (Colombia)/RConn2 -- Line115/LConn1
  PQ48/LConn1 -- San Mateo (Colombia)/LConn1
  Line117/LConn1 -- El Vigia II 230kV/RConn2
  PV22/RConn1 -- Termobarrancas/RConn1
  Acarigua II 230kV/LConn1 -- Line122/LConn1
  Acarigua II 230kV/LConn2 -- Line84/LConn1
  PQ15/LConn1 -- Acarigua II 230kV/RConn3
  Line143/RConn1 -- Acarigua II 230kV/RConn1
  Acarigua II 230kV/RConn2 -- Line159/RConn1
  Barinas IV 230kV/LConn4 -- Line159/LConn1
  Line119/RConn1 -- Planta Centro 230kV/RConn1
  Line121/RConn1 -- Planta Centro 230kV/RConn2
  Isiro 230kV/RConn1 -- Auto50/LConn1
  PQ64/LConn1 -- Isiro 230kV/RConn2
  Isiro 230kV/LConn1 -- Line119/LConn1
  Isiro 230kV/LConn2 -- Line121/LConn1
  Auto50/RConn1 -- Isiro 115kV/RConn1
  Isiro 115kV/LConn4 -- PQ50/LConn1
  Isiro 115kV/LConn3 -- Line145/LConn1
  Line145/RConn1 -- Coro II/RConn1
  Punto Fijo II/LConn2 -- Line153/LConn1
  Punto Fijo II/LConn1 -- Line150/LConn1
  Line150/RConn1 -- Punto Fijo I/LConn1
  Line153/RConn1 -- Punto Fijo I/LConn2
  Punto Fijo I/RConn1 -- PV1/RConn1
  Syn10/RConn1 -- Punto Fijo I/RConn2
  PQ56/LConn1 -- Punto Fijo II/RConn3
  Line142/RConn1 -- Punto Fijo II/RConn2
  Line173/RConn1 -- Punto Fijo II/RConn1
  Isiro 115kV/LConn1 -- Line173/LConn1
  Isiro 115kV/LConn2 -- Line142/LConn1
  Coro II/LConn2 -- Shunt3/LConn1
  PV38/RConn1 -- Coro II/LConn1
  Gen. Barinas 2012/LConn1 -- PV19/RConn1
  Uribante 230kV/RConn3 -- Line175/LConn1
  Line175/RConn1 -- Gen. Barinas 2012/RConn1
  Gen. Barinas 1/LConn1 -- PV20/RConn1
  Cabimas 230kV/LConn1 -- Line176/LConn1
  Line176/RConn1 -- Gen. Barinas 1/RConn1
  Line2/LConn1 -- Malena/RConn4
  Line1/LConn1 -- Malena/RConn3
  Line/LConn1 -- Malena/RConn2
  El Rincon 138kV/RConn5 -- Line136/LConn1
  El Rincon 138kV/RConn4 -- Line135/LConn1
  Planta Centro 400kV/LConn3 -- Auto37/LConn1
  Line85/RConn1 -- Planta Centro 400kV/RConn3
  Line91/RConn1 -- Planta Centro 400kV/RConn1
  Line90/RConn1 -- Planta Centro 400kV/RConn2
  Line144/RConn1 -- Caruachi/RConn1
  Caruachi/LConn1 -- Line6/LConn1
